simulink model "kuka_sim"  (R2018b)
settings: Solver=VariableStepAuto  StartTime=0.0  StopTime=20  RelTol=1e-3
model workspace (MAT data in the model file):
  F1 = sym
  F1.s = 'symobj::fromString("eJzVGktvG0V4/AiukzQE1CoUUtVQ4NILFMGhFZWD85CluAEaUIRUlo137Czdh7O7TuIgoYB4lQMcgN64IuWIVHHrtRI9cEA9wKXwA5C4capkdmbX8XietteNEksj7zc7833ffO+Z2QwAIA3A3q3wP5tJjYV/xadB9MuEz6fi53AMyKPmt3zd9826g7t73l9EbRuanlHY0j1TX7dgwdFt6BeaPjQKplPwW7a7/uF807ZbZQM6gVkzoQdImmkKZxa1DdcyqDEiHvF433IDqv8x1PzAsMx1TG8cdH8nUfNhcK1lz1mm7kM/WtsZgsY9YvzIBHYaNaFM+hPK83F/yEjxfPycooQ0jMAyqM27Ni0sLMiKHnjmDuZRRDNDPf9K4MhS8BhF43HUFnYaHgwF5zqLJkRLBcVnuvgw7XNdfIh+NnxfnOqi6cGJ1pQ2DdxP0p7g4KmEfRnA/Jh5JDwpMZgMxUsOtZLrBKG6Ed5n4/7psH0V8QAMic5OoKbBUEA+3OTpbaWJ8TJ6NvRA56yjQyfLw6WZNSAZE/Fi6bstzfUkPGO70eBmU7ewLGfjd6m4ZSiZp1BnO/xJ7GhG5SOO2/ApWjw8T6l8OFqf7mDzUenFgvEqGRokfFayrgJnLC2v7AC+Rq8/zfPpkt5oWC1mfTK/fZHDFx13SPng5jYYGozN2ToaVJzp4u7BSfJwgYJnOTyK4qBqbYzPhglkselUgYLmhIIOIxNOXJpWxJth4LPxM9JTJ+ZMEuvLR/x27KQbl9rtT04ANi7RMnuCWhu2iSDCxfRz8iHutwEjiwlJjCTHnVLI4NVHIFMV/EIXHDnufm1MVvyg5/E6dMKUEZu2XL9kvufiml+paNdW3y5fXcLvRTkxz7F3wt72RHmQ5oeEn+TZ007Ep0yWSfyXt+ZH7ccy+I0h5jM6rFSWu+WJWC8q3xtF3MU5tVQNq+R11xog5/WrP5xvdAPXSyRd3L9WWab7cR5YsKAd125MjWnj3UMi+yLhBQpeOmb2hDZIY296phPnAXLsODUW1e5TDtwOS9sAHoi41/7IPMT4usHSGJUdYnsIeQNAUXPqXt0HqjrY0506xLz21Lzp+B+I6501Cp7irJekJ5LpUbchEn5XYgP95siUQo603Eh9H3VZMfGS2IOI5NZvTi3x/AxvE+R+xvjFusvE74H2cr7roTOKGWIM7a+ymFtXyLFwzPSM42qoZz8+rOrHP3j+ItLHOQo2JTEtsrmmw9v3qvRC+x29ruOkExzbqy70qlFs76duKg3gR3nU0LHPxSCM5rhbKuskdUbjmMkex+sbEEWmnnFzQL5nwfUcqt/LV1fRO9F+JUfhle1XyHHzEp3QOjgt0Zer8KMpIK4ZRGcg9Djar7FsNAfW9QAZtHBei8PbMOfA3JqrVEUnBdyzIF4OIefjvBG0GpCn87AihXV80p6oVmfkRdgSbS+H6U/bCec3+swp3PpgFYOKfOEHdhCdX4vGRfZ3cHsitGmVXc3y7MqI7jY6OHLcPFTVfRitRRZnFyS83JS8+1riN6q9CpMXkN0tLq/MrbL80rGcpDNIDJpR+MrrktyFc6MHg6bnMPyheSe7YM+7b/uU7aDrkNaaNU+vctaaBr2/ywTPotj4vYQWtjHPbTqcfSst21sU/EOfNJPEX3wWVHWdLegFWuAqefxiwNgpm3vY9ccw8ZKJKY2NsExW3lPmLitw73Pe8+4o6fyvwimqbei98Z6Cn9U+c8M7Cp7eV7zXjoENkHCScwoS/kDxnneHe9TkQvoGrgnm8aPUZgMK3hqCruzuQjb3jALm0aK/fWD2gsSdCzn3yhDrIvw10TOJt0jBt3lrKJlG58yQuZ8HUezofIOSVsgE3d1NRzK5dKns1EzHDFoD5IgrgHPWReAhx/4yAh9g9hKGWasB8b6PqYNrGJTmRPYbjYiGSCYXODlbtu7rCXLyaxR855DjTlJ4j4In1bk59VBhB9gnTH8Xemw9NIo8fTdBnr4r0W2eo1umPifWJaotc8Q7mp88HSMy/HHIRsn9/HNdng++P8gQfbE/Cf0m2qvZTUv0rUE96j+o39vt9sfh32doHvrYrHr7m3tg76MyybuSXsNqxmeUIpnfB5x976b2smYY+Hs7kp+tDj/owub6w92XbvzzU+vnVz7/7cuNIKf4Duq+hNfovqnhbscfWjJ3HCE/gML3HsVbs8Mb+ljkvzv7/75V/rE+8d3+pzd/f/C3grc/FHyT8J8U/NcAcx8MIk8Q6ZeJvee1NY0X9xeX55b+B5OCZnE=", 2)'
  F2 = sym
  F2.s = 'symobj::fromString("eJzVG2tsFEV47q61FEoFA1QU5BQFExKNTfAHRNLSBzZpwUgRfOCxvd1eV+92r7t7bQ9fNTGK/JDEKJr4iD/0hzEmREH/+PiBIUETjYlIhKCJJD74gSGCBjHWndm93tw3szO3t0dDL5l0v9nZ7/2a2W0CIRRHaHK/+7chEWt0/3Rch7xfwr1e5F+7a1AzHnbRVmxbzxhkuuJ+Ox7jmm6pyTHF0pWhrJY0lJxmJwu2piZ1I2kXc+bQI92FXK7Yp2qGow/rmoVomnGAswGPETOrgjVBPJL1dtZ0wPxVeNiOmtWHCL25qPybj4etOVuLuc6srtia7cm2lKLxJbW+bgpbjEegTqpTys3+vMtIx0r/OgaUVIvCEnh0mzmoLKLIAcWx9AnCYxDNBLg+SuFoAHAjoHE1Hj0TeUtzFWcavbqGRUUd15fxEdoryvgw/Qb3fkdrGU0FTixTXFfJPE17HgfPgDuXQMyPeY6GWwQOkwC8NOHRZRqOa26M90Z/foE79ng8IFVgszl4pDRXQbY2yrPblgLBy9hZVRyFI0eJTgMPV0ofRoI1Hi9ZZXcxZVoCnonfpLTRgpIlulzm34v5IwF0HsOTU+5P4EdtshgxzLwNaPHwXCuLYU8+xSDuI7NLVvOlZGjQ8HKBXEnOWqivhhCxBuWP82K6S8nns0VGPlHcruLwBfMOrR8yzDxDg/G5nIIXdbSVcVfgpHlYA+BlHB6D8qBMNiZm3QLSWzDSSEJznoQOoxNOXlogyTe1wMv9a2ynUs5poeRr9vgt+Uk5L01NPT0HsXkJ6mwhkI34hOPhYuY59ZDM5xCji3mCHEmvWyTRwdrLoFMZfEsZrDvuan1M1Pzg67kZzXBLhu/aYvvS9Z6Lq3vLQGrr4L19mzeR+0E1sZnj75S/TQbVQcgPDV/D86cJj0+RLqPEL0/myx3HInhjDc8zNhwY6C+3J8F2kcVePfIuqaldabdLHjKzIWpetfYj9UZRSb9E0yXzOwb64TypAz1ZLef3bkyPmSO7h0j+RcM9AN40y/wJb5Aa77F0w68D9Nq5YC3u3VsNbdxtbR1tWsWV/kfXISbWVZZGvfyQ+IPLG0KSnlOxMjaS9cGWYmQ0wmtFzxv3/6LgfmcHgFs58tL0gnR6pfsQDd8n8IFqa2RMokeoN9reV7qumHxJ7UGC9FZtTe3ixRnZJojjjImLIZPJ36H2crZp4TOKNmoNjFdRzs1I9JicZXYmedW1s+0fVlUTH7x4CbLHCgDrgpzm+VzB4O17ZXaBcQflmk02Ibk9bWpW2svt1fRNXSHiqBkPfOzT7rjZnEwLdR2lz8jPMt2TfP2ohjNTxbpOJN6zkH4O9+99mwfxvaD9ShPAK9qv0Ou6BTaBNlgssJcpiaNWFNwzBJ2BwHUwroluUoaWURzs0IHPFTm81XIOzO25utL4pIB7FsSrIfTzpG44xbzGs7nbkWoZctIeqVdn9EX5EvSXmYyn8YjP56usKdz+YJCAknphOznHO78OWuf53/Tbk0CflvnVMp5fqd67jRKOJm4dSiu25skiyrM9Al6eF9zbK4gb2V6FqQvY73r7t3QOsvzCXE7TCZOD2iSxcpegdpHaaGlOwTIY/vBz88tgxb19Veo2rBzCXnPYUtIcWeOo8ree4jkoN74koEV8zDILBmffCnW7H8AvV0kzSv4lZ0Fp0xjTLCflmFIenw2ZO0XPznT/UUu+ZHJKfsRtk6XvKZvWS3C/y7nPe0cJ678MZ1BvA/fGkxJ+BqusDdskPD0suZ+aBT5Aw1HOKWh4l+Q+7x3ulaYXOjZIT9BNLoU+6wB4rAa6oncXomeXSmAeLfjtA7MXpN650M9uqEEuKl4jXdN4OwB8kCdDl66WzgyZ9/PIyx2lb1DiEp3gd3cLPJ2sW9dnDOuG7hRD1IgNiHPWReGh135Uhxhg9hKqPjyMgvd9TB88TEBhTWS/0fBoBOlkDadmi+TeGaEm3wngT2c470SFJwHcIq/NsX8lfkBiQrd3axbbD9WjTh+JUKePCGzbzLEt059TcgX1lk3UPchPM8wRCf467KP0fv6mMs/T3x8kqDk/niR7tXy24J8ZBn2r5K3LFbKcbxLIXnM01Z5STQcJ9Pid4N4xxHmHMJq6A+Jj3wflzXHJh5AEl60bkG+fBv72soKXBwS18BiAT8jopk0b4sfPTO+HpqamnnD/POOOxjmI/fnfcdHrHy+txx+gnDq8Ob5w4oL60M49B8+Ovb4KfPcl4//7CPaCMtHwyRA8HAfwTxxctPwTiNLXt489ePyzg/s+ePOV1emRtQdeqUJ+5jzF9bOUSpyX4aNquqgyzmQyn5HIKLQxoNVYg37rZXOa590lnnHSf3tPy3sf//7Nk7teuOHzX7bbkyH1w+OZpuWUaOGXtPqPo3uPHt74/uJLX5398Ix9yKdFr3+qtN5NtOiANRJ757Uvkl//vfX0mueW/ICi6fPkZdJnocQz/qj37ot9h25dfWLbG69eGDp3W9s5FE2f0N+E+uTkIKE+QQzC8/8wdcCPz3ZefP4WMs/R8M9AnnFExfb2t1bfnlz6ycVTS8aG7j+75MWQORXmwj8BfClEfiK9cIaAwhx5vo65R6gLNDOxErVm/BUxNmj4D4H9wvo2Df8H4NMR/PnXShj/c0XN/gB0iV2wZt//p3Y/jUH9QbvQuGqpgTQt2OOfR5z95crUDnyuxuxte/s7N/0PY1GX6S==", 2)'
  F3 = sym
  F3.s = 'symobj::fromString("eJzVG21sFEV0rtdaCqVWEQEBqaL+URIpIAlfKbQFG6igFEJM9Nzebcvi3e51d49yqAQTQoREiaIEfxj9YWIg4YfGkBg1MTEhwY8/xg9UQDEYlagQSIwose7M7vXm3szO7NwehG4yuX2zs2/e93szs5dECNUhtPOA91ufTDR4Px23If9Keve3BPfeGNSEm1N0NMcxBk3SXfG8Hbdh3bAzbVs129D6s3qbqeV0p63g6Jk2w2xzijmrf0tXIZcr9mR00zUGDN1G9Jx1AGc9bputbAaMCaORjHeylgv6b8DNcTNZo5/MNx6Vr4m4Obq7vphbnjU0R3d83qZRc3xCja+ZwCbjFiqTaEK5K+j3COmYHdwngJCqEVgSty4rB4VFBNmrubaxjdAYNmcS3B+ncNQDuAHMcSNu3dvytu4JzjJXGjpmFXVML+Mjc88q48Pz13vPO1rKaCpwYp7qjAzpp+eewMHT6/UlEXMx79Fws8BgkoCWRtw6LdP11I3x3hH0t3rtOZ8GlBHobBxuKd0TkKMP8fS2tkDwMnrOaK7G4aM0Tz0PV8oYQIIxPi1ZbXsxZdkCmondpPShgpYlspwRPEsELQlknsCdI94lsKMpMh8xrbwD5uLhmSrzYZ8/zSTmI9NLVg+4ZOag4ZkCvto4Y6G86hV8DfJfx/PpTi2fzxYZ/kR+ew+HLhh3aPmQZuWZORiby2l4UMeUMu4KnDQN9wJ4BofGsDgo443xWS+BrCyYaSSZc4JkHkYmnLjUKok31cAzg3usp1LMaab4a/LpLdlJOS6NjDw7DrFxCcrsJsAbsQnXx8X0c/Ih6c8hRhYTBDGSHneLRAYLroJMZfDdZbDmuKPamKj4wffjB3XTSxmBaYv1S+d7Lq6utb2p9X2P9Dy0ijwPy4lNHHun7G1nWB6E9NDwzTx72ubTKZJlHP/l8Xy1/VgEr6jifUaHvb1ryuVJuF5kvleLuEtyamfaq5L7raxCzouqP5JvtAypl+h5Sf+m3jWwn+SB7qyeC2o3psbMkdVDLPui4W4Arxpj9oQXSA3rbMMM8gA9djwYi2v3FlMf9kpbVx8VcaX90XmI8fUMO0et7JDYg0cbQpKaU7MHHSSrg23NHNQJrRU1b13wi8LrnU0AbuHwS88XJtPr3YZoeKPABqLmyIREjlButL6vd1kx8ZJag4TJLWpO7eT5GVkmiP2M8Yt+i4nfSms5x7LxHsUUagz0V1HMHZTIsW2M6ZnEVU/PTrBZFcU/eP4Spo9ZADYEMc23uYLJW/fK9AL9DvI1lnRCYnva0u20H9uj1E2dCn7UhBve9ml3vWhOuoWyjlNn5MeY7Em8flLHkali3HIkXrOQeg7X7z0P9eFnYeuVRoBXtF6hx3UJdAJ1MFmgL0viRy0ovGYI2wOB46BfE9mkTH1Qc7FBh75X5NBWzT4wt+bqTOOdAu5eEC+H0O+TvOEW8zpP515Fqg+SnfZYtTojL8qWoL1cS38ajvl+PmJO4dYHfQSU5AvHzbn+/nXYON/+Rk9PQm1aZlczeHaV8c82SjgauXkorTm6z4soznYLaNkjeLZX4DeytQqTF7DdrVyzdnkfSy+M5fQ8KjFoisRXlgpyF8mNtu4WbJOhD783sQxWPNsXUbaqfAhrzQFbS3N4rUOV12KK5rDY+LJgLmJjtlUwOetWKNsDAH4l4pxx4i/ZC0pb5lbddlOuJaVxt2LsFL17reuPauIlE1Pym70yWXpO2bhYgvsQ5znvjBLmfxnOsNoGro13Sujpi5gbNkhoelzyPDUGbICG4+xT0PATkue8M9zrTS60b5CaoIvcCm3WBfDWKuYVnV2I3p0mgXlzwW8fmLUgdeZCv7usCr4of411T+PtAPC7PB46jUxpz5A5n0d+7Ch9g1InkQk+u2v1ZbJoUY85YJiGW1TIEcsQZ6+LwkOPPVoDH2DWEhljYACFr/uYOniAgMKcyH6j4c8RJpN7OTlbxPdjMXLyAwD+8BrHnbjwTgA3y3Nz4orEDohPGM523WbroVrk6WMx8vQxgW6bOLpl6nOKr7DaspF6BulpgjEiyR+HbZRez99Zpnn0+4Mk1Rf40+i8zYi3VstnC8GeYdi3Sv64XCHrVo6DdTmhwzHImpPpH0rNQwI5fynIQV8hzvp2KNWeylhuVJzwGcQZ0DgX4mPPoPLWMOfjSxr313zc+DvPinGPSnim4ZMyuactB+LH74yuvUZGRp7xfnZ5rWEcYq/gm7HI41Glbcl0RnKOJ99UhiitYuwpAP8E6CiU6PCcHr39Uve61eOaH3xx0sn/Pp+45EgEOsJs4HsAf8fRDw2fBnQ9XaILf3j5xq5Xj95/tPXs6wsnH7pv0o5D4Bs8FbpkdiuyC/rZjwD+RsHeoCygjk5QuBpi0P8NkCn+7GTU5i5ruy6Yu6dfeL94uHPCwY+i6FrEwxkAX1L0Pxo+D+geLtGNN2S0PY0vH31v7tIvFuy33lh7tgfQDeVVjexp+C9Ay44SLV5iQWcvzvri9NDeFz5eccT499M/jyM1vw1i7TyVWCuT5YmIeKLYflSblMn4fISYRMM/K/B7XsJvmI/K+JfZN4yj+JCH2AUuzN6e33/51h+WTT75fHLXr38fPBwhXjF1+iABhTT8o54j2nk5AvqbMCdE4IWCE7DGO6EiN6QWk2i6ahk3XUT5/FvHVi+c885r56fWb2zZ8oG7X5FGiV0lWhRw8XwUxq5a+mzkmBzYSJit8uQftY6APMM64g/F2EHDvwFdNCvgulKjuAtpEv3XgBf7afphzXKOwgXXeCr1fBBL5nFiSWL8VfDXauqHWvpU5BoKxMZa58lLMXBL6hwio8h1jmIOgHZ4WTGP0fC3NfIzqOdTtYvhjKzPKeAGez2J+rB8ie3vjqUHNjzauuThxu4zM3v2vYmfqeSiXyS5SMGXo+d5Ht1q9lRR88GxKnHjWwCfBTQ/VaIZ/yHlM+r63GuKNENZw3wqnAvFW+NAW4d6ng/gexT4OhFRFxJ/hPaTaFd4F34HdUpBVr+r+XIsWcnqjftj5Gcaz+0AVqljLoJ3744Rq2E9KuJXMYck4H87VHMIjQucX+A/UNcshirInomhsI6ZU72tJZbUTo+JhTF8AOa36RybYM6fZqc24XN35uxr5Zrlq/4HI4LjiQ==", 2)'
  F4 = sym
  F4.s = 'symobj::fromString("eJzVG2tsHMV51ufgOC9CRWLSBOE0KRTSFyYgNTxkc06iUJug4KIQ2l7Xd2uzcLd72d1LfOGhRFQVkCr90Tbwt6qEqPqrUB4C8gspVau0AolA0qqNq0SN0lZVVKmoSCCzM7vn++6b2Zmd3UsUn7Tyfrsz3/s1s+MCIaSHkINHw7+9BWNR+Gf4iyT6FcL7a+P7cAzpp5ff9E3ft6cd9rjj/RC99lu2VxncZ3q2OVm1Bh2zZvmDDd+qDNrOoN+suZOPjTZqteaOiuUE9pRteQTS7EE4e+n1qFutoDFJPLLxftUN0POr6OUHlao9yegtIe3fcnr5VvBgszZStU3f8iPZ1gAafwDju6awVfRK1Ek6pWyMn4eMDG+I7w2kpCwKK9Br1K1hZTFFjpuBZ88wHpNoFtD97wGOXgQvQjSuptfWmbpnhYpznW22RUUlw2vb+BjtG9r4KP3e8P3wijaaDpxUph67wp5D2ksFeMbDZwXC/bh5EF4mcZgC4qWPXkXXCUJzU7zr4+crw+vZiAdSkdhsMb1KVqgg39orstvOBsPL2bliBqZAjhadXhGukj1FJGMiXqrmgWbJ9SQ8M78pWXsbZpXpcl38zoivAtK5QR/OhT+JHw2oYsRx6z6iJcJznSqGI/lMh7mPyi5VK5aSowHh6yVyDQrGYn31asQalr9HFNNFs16vNjn5ZHF7o4AvnHegftjl1jkanM/VTDpoeKCNuwMn5GETgtcJeEzKgyrZuJgNC8i2hlMmCppLFXQ4nQjy0kpFvskCXx/fUzu1cs4yIF9/xG/LT9p5aW7u0GLC5yWss2uQbMwngggX91xQD9nzGuF0sVSSI+G4axU6uP0S6FQFf7kNdh13Wh+TNT/0fsm05YQlI3ZtuX1hvRfiGt05XnpwYteO+7ez90k1sV/g78DfDibVQcwPhL8g8qeZiE+ZLvPEr0jmSx3HMvjeDPM5G46Pj7Xbk2S7qGKvG3mX1dRiOeySJ92qRs1Laz9Wb8wK65cgXfZ89/gYfs7qwNaqVYt7N67HrLHVQy7/gvBWBG9fYP5EF0iLHvBsJ64DcOwSNJb27isca3/Y2gbWvIo7/Q/WIS7WKzyNbvkh84eQN0IUPafpTftE1Qd7pjNtMV47et6e+C9J7nd2I3iFQF5IL0mnV7oPQfghiQ+krZGGQo9Yb9DeV7quuHwJ1iBJektbU4uiOGPLBHmccXEx6XL5W2st57se3aMYAGNwvMpy7rRCj4MLzM4sr4Z29uPNqjTxIYqXJHvcgGBbktMin2s4onWvyi447rBcC8kmLLeXXcsrR7k9Td9U1IijfnrRbZ+hIMzm7LFU13n6jPoC0z3L149bNDN1jBsh8jUL6+do/77j/gn6Lmm90ofwytYrcNyoxCbYBqsk9nIVcbSCJPcMSXsgeByOa6abkmNNmwF16MR5TQFvWfaBhT1XsUx3CoR7QaIaAuezuhE065bI5mFHak2znfZcvTqnL+BL2F8uZzztzzm/nrKmCPuDCQYq6oUf1IJo/zppXOR/819PEn1a5VfrRH5Vib5ttHD0CetQ2fStSBZZnt0q4eU5ybvnJXGjWqtwdYH63baxnSMTPL84l0M6OjloQBErd0tqF6uNnhU0PIfjj85b3gY73v0kpW515ZD2mlOeWRbI2kM6f3cCnpNy488ktJiPeW7DEaxbsW6PIvjnKWnmyb9sL6jsOvssLygFrpLHH2nmTtncy91/ZMmXXE6pPxq2ycrvlH13KnD/SvBe9I0S138VzqTeBq+NDyr4mUhZG76j4On7ivelBeADEM6zTwHhHyjei77hXml6gbHBeoJRdiv12QDB+zLQlX27kM1do4BFtPDZB24tCL65wLn3ZJALxGuue4h3GMG/FclQtCutPUPu+zyJckfrDEqPQif0293KSCdbtuxwpmzHDpoaNeIeItjrAnjg2Ne7EAPcWqJiT02R5HUf1wdPMVBaE/kzGhGNJJ1sEtRsmdzfy1GT70Dwscucd/LCBxG8TF2bjU8VfsBiwvYPWB7fD3WjTh/PUaePS2zbL7At158DuZJ6yz7wDvPTj3NEQTyO+ihcz3+pzfP8+YMCeBbH0zxd8Z5hvdqI9wyTzipF42qNatA5DuvqA0kdOUmS+3nGv2+ztSr3fG9pc1qa+N1JMb4hIrHTh+I5t8E5i9LRuRXT4caUXar5Dlx/VvAG4dMErK3m5uaeCv/8kPK3mPC/+ExY6vGk03dU9oTv/obgjxT2S5JfZE8I/1WDh9MI/juYe5WmT2HZoE7psQmmU7owv+mY++T6Xz9y96t9ew4dKr68C53LE+kUwqcQfDaJVphAyHfX3nL8lRdPPfnBGycuVC4UBzRpYf2c0ZGLqH0Fwv9A8AUduRAtUSxiH4HwLIL/guCLiJenW7zQYva7m7d4S197qfmNt2+6+r2TD/07g9xJY1W5k9vfC3NSqeKysxRZ87FMD2cRfE4D1xmBfXHsJcWiKoez3jXM4aUKE56TQYfHrHoT2GJIxxY6eU18DqLu7o//AUDm23tyxP95hc1U/iCw2a0im2GeRXRgPB4goGa9PLP8Tw+885Wx684ffuGZWx4eIXrxiPKrsQTR8iCtnw68deTcJ8+6J766ZuiXv/jNO5r5VRX7An3d1tJXWhqyM986/od9YVaDB5xvsR/NasY+tA+u0+d17EXy+cYqBMv2TBJyxOZu5ohTXcKDa/FZTR5wntehm6YWpum/MvqTsOfJ6uezglqUOm/p5RIDfofqZu9aJ6DHO9LYu/bYrqPrN19zx10/vu+f8bo8c4+H+4n/5qhNuDeV8p2z58a9C+S7y72ncTPR6D015ZL5tk6fOId47kU8P9Himf6DxAnw+2N4afo59u1ZHVok3zpB0Q8ZQwj+uoZcay5N7jZk36dV9W29II/C98s1cMv6cB35PkM8fFMxl9tHnmZgYi8j8okE/AbGg/1lj9xfcOxL/WeZps4EveNmQa9trNa0IZy7ODsuzrf+h+CPM9Y+bD+dPKaqTxdz1AyEi+X1PHsjENeNOfjCtexidjtwuQevneiBwvnc/PFzxXdXn924+r3Db/xn5s33D5Pu9uLjmri6kXvRHocxnCO28P/X4dyrW1sgvEHHLpo9xWcKnejUjDx7Y5Am+kZsoG8oLO+mxXWXIqer1hppawnuNfYIeM4ap/+/NP6utU7Ee4s4p8Faolv7IB50Jly5Rtepdxq4cL0zvpbDfqI9qqy5D+dsnEcncuDalUNGVR7ZqIHrX2jut7PzxeXSb+WsO3DuIzljGuJC570M/J2XnY/YUNpNx3FnM7aNjWz/HMzJdIk=", 2)'
  F5 = sym
  F5.s = 'symobj::fromString("eJzVG1tsHFf1jteJH3kTB6ckpds2gEQAKU5cqQ9HDnZspbIbSN0qCirLeHd2O7A7s96ZTbIpD/NQaSACVaIRH3zQByAkFPHRVlWlSP2hKhUVP7Qp9KW0qAiKiFokhBDCzL0zm7177pl75+5Moni1Y8+ZuXPOued97tzNEUL6CFk+G/zvzxlrgn+THyHhJxecj0TnwRgyRA+v5ZmeZ1ccdrnr/hg9Tlh2o5Q/bjZsc7Fq5R2zZnn5pmeV8raT91o1d/HL081arXWoZDm+XbatBuFp9gGc/fS4362WwJg4Htl4r+r64Ppaenh+qWovMnrDpPPZQA/P8u9u1Q5UbdOzvHBu13E0XuTGZyawbfSIlUkyoeyKrgeMTN4cnRtASL0ILEePabcGhcUEOW/6Dfsk4zGOZg6c/5bD0Q/gNYDGJnocPFlvWIHgXGfGtuhUyeSODj5G+4YOPkq/P7g/ubGDpgsnnVOfXWLXedrrEDzzwbUcET7Cczy8XmIwOcDLAD2mXMcP1E3x3hhd3xwcD4U8kJJEZ4P0KFiBgDxrCdPb4SbDK+i5ZPomMo82nX4MV8EuE8mYkJeqeapVcBsSnpndFKylplllstwZ3TOiIwdkbtCLK8FHYkejKh9x3LoHaGF4tqt8OJyf6TDzUemlakWzFGjw8PWSeeWRsVBe/Rq+Buffh/n0lFmvV1vC/GR++3GELxh3ePmww60LNASbq5l00ORoB3cXTp6H3QDeifAYFwdVcxN8NkggM02nSBQ01ynoCDJB4tJmRbzpBb4+Oqd6asec9dz8hkJ+23bSiUsrK98cJGJcgjLbAubGbMIPcQnXkXzIrteIIIt1khjJjxtRyGD8CshUBX+sA2aOO6mNyYofej5csZwgZUSmLdcvn+9RXNOH5wt3Lxw5dNcsux+XE4cQe+fsbTkuD0J+ePhDmD2dDPmUyTKN/2JzvtJ+LIM/28Pzgg7n5+c65Um8XlS+l0XcZTl1qhhUyYtuVSPnJdUfyzdmidVLPF12/ej8HLzO8sDBqlWLajehxqyx7iGVffHwQQDPrjJ7og3Sms81bCfKA/zYYTCW1u4bHetEUNr61mURd9sfn4cEXy+JNLKyQ2YPAW+EKGpOs1HxiKoObphOxWK8dtW8fdF/El/vHAXwRmS+PL04mV7rNsTD90psIGmONBRyhHLj9X2ty0qIl1wPEie3pDl1CvMz1ibI/Uzwi0VXiN9avZznNugaxSg3BvqrLOZWFHLMrzI9s7ga6NmLFquS+AfmL3H6uAHAtiSmhTbXdLC+V6UX6HdwXqtJJyy2F12rUQxje5K6aUrDj4boQZd9xvwgmrPLUlmnqTPqq0z2LF5/xaKRqWvcASLvWVg9R+v3Q3ct0Htx/coAwCvrV/hx0xKdQB1sk+jLVfjRRhJfM8StgcBx0K+ZbAqOVTF9atCxz7UQ3npZB0ZrrqkiXSlA14KwHMI/z/KG36pbmM6DitSqsJX2VLW6IC/OlqC9XE1/OpHy+XrCnILWBwsMVOQLz6/54fp13LjQ/i6/PYm1aZVd7cTsqhS+22jjGEDzUNH0rHAusjh7UMLLacm970n8RtWrCHmB2t3M3OEDCyK/MJbzdHRi0KjCVyYkuYvlxoblNxuOwB99bkMH7Lr3w4Sy1Z2HtNYsN8wiMtc+0v25neM5Ljb+SEKL2VjDbTpI3wplexbAjySkmSb+srWgousctxp+wXeVPD6oGTtlz17t+qOXeCnElPr9QZmsfE85cLsC9y+R+9g7Spj/VTjjahvYGy8r+FlImBvuUfD0RcX9wiqwAR5Os07Bw19S3Mfe4V5rcuF9g9UE0+xUarM+gI/3QFf27kL27HUKGKMF9z4IvSD3zoV/dn8P8+L8NdU5j3cSwE9ic5iyS+01Q+H9PAljR3sPSp9CJvTd3eZQJrfddsgp247ttzRyxH6CrHVxePixT2fgA0IvUbLLZRLf9wl1cJmB0pwo7tEIacTJZDeSs2Xzvi9FTr4FwOevctxJCy8DeL06Nxv/VdgB8wnbO2U1xHooizz9fIo8/bxEt0OIboX6nJtXXG05wN2D/AzBGJHDx1Eb5fv5mzo8X95/kOOuRf50me4GgvVq9WozWjOM26sUjqs1q373OFiXMz6KLsUmXl8qjEMa/Nz+INHByxK5voLT2peUFrz3MkF66aXC3kLJ9YmERxVOqcw8m/XpyDz2JqWJyQzBR/eado17k8OxJhmOPUShDx5+QzL2dQC/RbhecWVl5WvBv+9QvgaJ+In2uCUeT7p9AdMRD7+tkHvcHDE98PBFDdm9BeA/I3BS/bOcH+i/UGKGHGsDaeWi6VdjOn6lI1v8/XHdPRFtnOafewfAxzTkAXX0V4XO/qIho0hnezCdQZ5ldHTiKfTJPyriKMLv3ja/SWX4fkb6h7p4R4OHiwo9YvJOyte/EdyafrIvSz/5X0Z4/gTgdzV54OH3NOn2WkdA2+5Vp9DW3lboVGZr0LbeRPji81zQ33fy3AtPPjzzmZcGX3xm4ic7tg/vfYGo81xS37/QDRtbAR/1Nh9BMU5O//3bn7p05ulPTj+0u/LYhufWgj3oKpm8yo2FdUhMnNmnG2egXP+jGZt5+BKi/15t6bWM/BHyoOOPUDbvAd2PJpeN8WEA53XsN4HdIPFxPMv4+KqEPqz9LmjYDIx576awGRh7NeIn009WcuLxDmvywMObAHxTwhiWgn+Bh2ENXcK5b5Locm0KGV8AvkONnPnOUPDnjYH8U7P3bJ0+/8SeY/aR4WeJXo+D2WNiWnrxHZU1T+tUmxZ9oblt/McPPvqNb32fbP/9T2d/9ZtfaOYSzDd42mMp9ZyYbxLqgx//dX78xPCFx4NvPfhOPFGfGNacZ1Z1nKx20cFzCcz1gfZc6Y9lfsd9XgoOxW/UYJxn68IVBsbW+Nj6RRz+DwAMa7JjAMb6gcRzJXp+KevHVT02D78P4H8BW96vgQv2MKBmNaYUepDJWtFDG3CvH6yHpT5FtGRv7L5CcdvhefxBc2nH+SNnb9y35ZY7ztz5t/4e/F4Wt6W09OSB5ngevjXDuHw4RT6B9cOtAJ7XwC2rY3T8D+uPY2PGudmLp4LvSPA998DIOfqLqDS5HMoW7Ns37lDgzqq/TjxfTR/A+m84317jkaIfF2QJbU8lW37srmxsTfCHT4DxOr0t9Hn47hTGX+k6ANGz46RrOyp5wH3R/5TkKxWuSXl+UvZtSWsQaNPHEJ7j7Gy9pp8i6ynjyDqzUdbQHbQbuF70VcLZSe7x17+77R8//9muM7/+YMsrm8sp+4m8Di2iVxPsAvCnAexp8t0eO9h7bDXAPpuueNdrv5x2/UInxihqAfg+w/hCClqKdb8u2WmuuxhzGnwo1gyN+zT4ALowqhp8vAae/agiv2nkM8FGwL4QrXVEkMMMsP9Tp6YT9AZqAp0419UjYGvVWdXWGusU6PoKD2vU1qq1LePzKfiCuMZS6JRfp4W/M0pTp0ObVcVWmV9CO9PAZYA5GWAvpk68MMA+P8PUmBOMU3cisbrHWGzA38/BuK/Ttw1I5JHivabWujDUP7YuHBcPdWs4Hg/4nZsxksJHtwJ4SWP+MHbkM8S1nCJWqPKS6n2DTi7RkT3McfemsH+ox4dT4II1rwVgnZoXxrFHepe9sQfAp5E5CnuDby4cpb+JEPYlz8wdmP0/qpZvwQ==", 2)'
  F6 = sym
  F6.s = 'symobj::fromString("eJzVHG1sHEd11ufEdpK6IXJkQhLFbdoI1EJVJ46gUSK7tmPSxk3UmDQEwbG+W1+X3O2eb/ecXCKiVEIRRQIEpVWKkCg/+EGlVqpa+o8fCKlSKfxBlFYtpAopKoqiUlokKGkxO3N7vrk3b2d2dtdRfPLq7u3Ovnnzvt+bXecIIV2EnHsi+O7OGauCr9FPkeYnF/weCH8HY0gfPbyGZ3qeXXLY6Y7rw/Q4adm14tCCWbPN2bI15JgVyxuqe1ZxyHaGvEbFnf3GRL1SaRwoWo5vz9lWjfBzdgGc3fR42C0XwZgoGtl4r+z64Pxqenh+sWzPsvnWkPbnJnp4ln+kURkr26Znec21beLm+C03PjOGbaRHJE/iMeW28HxAyOj28LcBmJSEYTl6TLgVyCzGyGnTr9mnGI1Rc+bA75c5HN0AXgXmuJkek6eqNStgnOvsty26VDK6uY2Pzb2tjY/O3x1cH+1vo+nASdfUZRfZeX7utQie6eBcjggf4T4eXidRmBygpYce467jB+KmeG8Jz68Pjm83aSBFicx66ZG3AgZ51jwmt0N1hleQc9H0TWQdrXm6MVx5e45IxjRpKZunG3m3JqGZ6U3emq+bZcbLLeE1IzxygOcGPbkYfCR6NKiyEcetemAuDM8nVTbcXJ/pMPVRyaVshasU5uDhrZJ1DSFjIb+6NWwNrr8Ls+lxs1otN4T1yex2B0IX9Ds8f9jhVoU5BJ2rmHTQ6GAbdwdOnoY7ALwFoTHKD6rWJthsEED2150CUcy5VjGPwBPEL61X+Jsk8NbwN5VTy+es49bX16S3pSdtv7S4+EgvEf0S5NknwNqYTvhNXMJ5JB6y8xUi8GKtxEfy4wYUPBhZBp6q4NvbYOa44+qYLPmhv9eULCcIGaFqy+XLx3sU18Sh6fyRmQcPPDDFrkfFxD5E3zl9OxcVByE9PLwB06dTTTplvExjv9ial9uOZfC9Ce4XZDg9fbCdnkTLRWV7WfhdFlPHC0GWPOuWNWJeXPmxeGMWWb7Ez8vOH5s+CM+zODBZtiph7ibkmBVWPaTSLx6eBPDUCtMnWiCtOlyznTAO8GPXgLE0d+93rJNBautbSyzu1D8+Dgm2XhTnyEoPmT4EtBGiyDnNWskjqjy4Zjoli9HakfN2hd8kOt85BuB+ZL38fFE8vdF1iIePSnQgbow0FHyEfOPlfaPzSvCXXA0Sxbe4MXUcszNWJsjtTLCLWVfw31q1nOfWaI9ikBsD7VXmc0sKPg6tMDkzvxrI2QubVXHsA7OXKHlsA7At8WlNnas7WN2rkgu0O7iulSQT5tsLrlUrNH17nLxpXMOO+uhB2z7DfuDN2Wkpr9PkGdUVxnvmr09Y1DN1jBsj8pqF5XM0fz/wwAy9FlWv9AC8snqFHzchkQmUwUaJvFyFHfWT6JwhqgcCx0G7ZrzJO1bJ9KlCR97XQGhL0gdGc67xAu0UoL0gLIbw97O44TeqFibzICO1SqzTnipXF/jF6RLUl+tpTydT3l+NGVPQ/GCGgYp44fkVv9m/jhrX1L+l3ZNInVbp1RZMr4rNvY0Wjh40DhVMz2quReZnJyW0PCq59h2J3ahqFSEuUL3bf/DQ2IxIL/Tl/Dw6PmhQYSt7JbGLxcaa5ddrjkAfve+mNthx7fsxeau7DmmuOVczC8hau0jnZw9Hc5Rv/JFkLqZjNbfuIHUr5O0TAH485pxp/C/rBRVcZ8Gq+XnfVdJ4XtN3yu693vlHEn8p+JTqw0GarNyn7NmjwP0L5Dq2RwnjvwpnVG4Da+NzCnpmYsaGLylo+prien4F6AAPp+lT8PDXFdexPdwbjS+8bbCcYIL9lOqsD+CFBPPK9i5k925SwNhc8NkHoRbk9lz4e/clWBdnr6l+83hHAfwCtoZxu9jqGQr786TpO1rPoHQpeEL37tY3eXLPPQecOdux/YZGjNhHkF4Xh4cf+2IGNiDUEkV7bo5E131CHjzHQGlMFJ/RaM4RxZM7kJgtW/dXU8Tk3QD+1XX2O2nhcwBep47NxkcKPWA2YXunrZqYD2URp19KEadfksi2D5GtkJ9z64rKLXu4a5CePugjcvg4qqN8PX9rm+al5w9y3LnQnpbmxXuG1XI97BlGPavUHFepl/3OcTAvZ3R4Nqs5hfPz+d38vavA2v5IkFp3Pj+SLxbZM3ZR8elVCc//hNOxC64V0iGbS6iz5/M784zEaB1S4dSkf2fcueA1SH+Ijz5/2jHuokROETjuJkShFwXXg/P8RbF2Hn6LcHXk4uLiN4Ovb1H6eon4CZ9/iz2edNoJJiMevqzgf9QaMXnw8CUJP/6K8IOH/4bAcfUgtLXhlq1F6UJavmja1bCOXenwFt9brronw4eq+fveBvBxDX5AGV1RyOzvGjwKZXY3JjNIMzaPjq7E1ck3FH4VoX9nHP/Ow+9npA9QNm9r0HBJIVeM/3Hp+hDBrWk3u7K0G9lzxLp4ePgdjXvfBPBVDVm9qdDJuDS8kUKmUNcua9APdQ3q1sUYcYCPg3SjbykOTp0/8evth3+64d383oGn3TrtJaviYFJdiOtDXtPwIWHuMUI09QHqYVK5Qp2+qnHv68vPSwM8O2/IalhVHirDu567d3UKG3sN6Cp9iIjpKi0k7WsPHR3rv+/CD9YU1l74b+MI0crZDLAHY2yOmos++DV16fRA8Pds8DcV/F3SnGsbwvfY6wLvbqjm2orIgodv07CN18G9twB4B1jH2dY6qON4+Tf3fnfjtVfeff6K98u+D58qxeAZErt2Zxi7jMGYeHT5shlcV+VtMj0EPO7wP3HokvnKuH41jv4m9JEq/WS843WKFolLOvW5j049uefiW//7zFP/md75kwu0v6Njh3ctk/yHM5Q/7BVuIhrxWtNXbOPG9mraFZK772rl7jy9Z1r00hdkAtd5uuVLzwSOlGSTX6SN8RryQmN8XFvQoRnLj3nZjaVY/1UEV1J+wHzzmoTO61VbyPJpHTzvyXT5d9zn98GheMcS2gzb1ygxUMjnZb22KPwfABjWCccBjNWosddK9Ppjsp6Rjk28D+B/A127XwMXrKtBHWUcVshBxmtFn4fhThrj30N0Pba/jaGj0G9kIDfjELj+LwmvVbjgPhDWQ4tT06jsB8rweHKayZ8z9GswJsS9F/ppRQwwPqshk0HJWB092RoTj24d/rGmzvM0rdagvzcjOUMaVHW6ZO1Cfq27LxCVL2L7dfzYUc34IMkhtPIRzD8mXC+zW35NluJepH4dybJ+hbXTZk3Z8TCs5Tdq8BjWP2cA/AUNmxnmxmbZK6I7N0t1UunsSM8zG+7sf/TKM4+MvzOyQPTyF0W9b+zQWK+qFySlO+Ne0FlNHw/1J3a/LKQ7aXzh4wJ8fyRNTfUxEgMT1lTG6uS4DFB703/d0AF/RcPOJyXzptjf6KBBd5/zsoQ3urm1Yr9DS4aQrocksUIzhhkPIrhi90o17Rza5gDR6KGBudZp6gzSB9qN7EHrxATB38L1LPXAAudJntvwwdUX/3Di+X/sevKfvUdffYWk682D98OMxzXlIMuPkvqWLyfXS9irNb4Ixuv0Kr8njydp+mgGfBYbPJNgPJYi7kFd1JEp6Mcad6ag6y4A79XR65Q+AeZoP9bAtSDxATr1HbS1NPsmUMbYvkka/7Mc+XopBa9+mKF98Dl3Cj+F7qEmzC+VOfanU9AFa50s90DPApjPa3VjKY/nAoD3ZRjT0tR6P1tGv6xBl+BLP5/cvynrWR1fuR3AL6TgF3hvx3g6hU5Am3hWordJ8k0e/nmK+Hoe4Zfwbsf2/DH6TpvwXsn+g2NT/wcyZPj9", 2)'
  F7 = sym
  F7.s = 'symobj::fromString("eJzVG11sHEd51mfXdv6ctGlDqNuYpPDSCFEncdpGLQ62YxnZiSFuCJXgWN+tnaV3u5fbPTtnq22oqlBaiUoEDO1DeUBUgoeIhxR4gCekolIQVDSFAqFKQ0tLVFD4EaUCmZ3ZPd/cN7MzOzvrKDl55ft2Z7//v/m5HEKoDaGTS8H/9pzREfwbfD8KP7ng++boezAGdePLq3um59mzDrnd8rwfX/OWXS32zZlV25wuWX2OWba8vppnFftsp8+rl93pzw/XyuX6WNFyfHvGtqqIptkGcLbj65hbKoIxcTyS8V7J9cH96/Dl+cWSPU3orUHNz3p8eZZ/uF7eX7JNz/JC2bZSNH5Gjc9MYTfiK1YnyZRyW3Q/YGRwR/TdAEpKo7AcvobdMlQWUeSE6VftE4THOJo58P0FCkc7gDsAjR58jZyoVK1Aca5zwLawqGjw5iY+QntbEx+m3x48H9zQRNOCE8vUZhfJfZr2Wg6eieBeDjEf5j0aXidwmBzgpRNfQ67jB+bGeD8Q3d8YXI+FPKCiwGZd+MpbgYI86zjPbodqBC9j56Lpmxw5GnTaebjy9gwSjAl5KZkL9bxbFfBM/CZvHa+ZJaLL3uiZEV05oHMD31wOPgI/2iKLEceteIAWD8/7ZDEcymc6xH1kdilZkZQMDRq+RSBXH2cs1Fe7QqxB+dt4MT1kViqlOiOfKG4/xOEL5h1aP+RyKwwNxufKJh40uKWJuwUnzcPtAO7l8BiXB2WyMTEbFJADNaeAJDTXSugwOuHkpY2SfJMGviX6ju3UyDnrKPm6Q34bftLMS8vLX+hCbF6COtsEZCM+4Ye4mPucekjulxGji7WCHEmP2yzRwZ5V0KkM/mATzBx3Uh8TNT/4+5pZywlKRuTaYvvS9Z6La/jQRP7w1CfHDo6S53E1sZvj75S/nYyrg5AfGr6e508nQj5FutSJX57Mqx3HIvhjKd5nbDgxMd5sT+LtIou9LPIuqalDhaBLnnZLCjUvqf1IvTGLpF+i6ZL7RyfG4X1SB0ZKVjnq3Zges0xmD1r+RcMjAB69xvwJT5A6Jqu2E9UBeuwaMBb37hscaz5obX1rRcWt/kfXISbWiyyNrPyQ+EPAG0KSntOsznpI1gdXTWfWIry29Lxt0X8U3+8cBfAGjrw0vTidXu0+RMNHBD6QtEYaEj1CvdH2vtp1xeRLag4Sp7ekNXWIF2dkmiCOMyYupl0mfyvN5Ty3itcotlBjYLyKcu6sRI9915idSV4N7OxFi1VJ4oMXL3H22AZgW5DTQp+rObx5r8wuMO6gXNeSTUhuL7hWtRDm9iR905BCHHXjCy/79PtBNie3hbrW6TMq15juSb5+wMKZqWXcfiSes5B+DvfvYwen8LO4+UonwCuar9DjhgU2gTa4UWAvVxJHG1B8zxC3BgLHwbgmusk71qzpY4eOfa/O4S3NOjC35xoq4JUC7loQr4bQ75O64dcrFs/mQUdqzZKVdq1endEX5UvQX65kPM1rvl9JWFO4/cEUASX1wvPLfrh+HTcu9L+V3ZNYn5b5VS/Pr4rh3kYDRye3DhVMzwplEeXZEQEvXxI8e1wQN7K5ClMXsN8dGD+0f4rlF+Zymo5KDtoiiZV7BLWL1Maq5deqDsMffm99E2x59mRC3arKIew1Z6pmgSNrG2r97KN4jsuNXxXQIj5WdWsOZ94KdbsE4K8lpKmTf8laUMF15qyqn/ddKY+nFHOn6N0r3X+kyZdMTqkcC9pk6T5l5z4J7u9wnvP2KGH9l+GM623g3PikhJ+phLXhPglPn5U8z18DPkDDOusUNPw5yXPeHu7Vphc6NkhPMEy+Cn3WB/BcCrqivQvRu1slMI8WPPvAzAWpPRf63XtTyEXFq9Z3Gu8ggM/yZBiyi401Q2Z/HoW5o3EGpU2iE7x3tzHUyd13jzkztmP7dYUacS/irHVReOix388gBpi5RNGemUHx8z6mD54hoLAmsmc0QhpxOrmdU7NFcn9GoyYPAPjHVzjv6MInAbxOXpuN/0r8gMSE7S1YVbYfyqJOP69Rp58X2LabY1umP6fkiustO6lnkJ9umCNy/HHYR+n5/PYmzyvnD3LUvSieVujy1wwrpVq0Zhh3VikcV66V/NZxsC8nfBRcjI29fzw/QL/bAWR7WVCDzsloerYTQ3M3TRPa9mXBM0iTfvYKn9YuJJBBRouZ5x/P9+eLRXK+cGX+tLy8vBj8ezS4OvABlJ9Tn18El+TcF6RDcu0sAWNlfZUvaz/9DrTlORSfq8N9vIo7Hx1g5eC+AwF890tsQcOvA/iiiv5Qa7zI/BDqiYb/kNAXeDSYtRziCy7ZN0/ryzT8pmDsGxz9xdmCx7vIFm8BWzyIIlt0IfYT+TL9/msKeoti6I5GDIlkelviy1B3Mhkhbhq+zIGT+FuWuYuGf5eRT0E9vKOh0/MSe11W4Ov3EvniYjZJDEG7J9GjLGZgH7Usyl9nRi8sBH+bg78zi5vP4FNUsvwFdUPBBvAVfEg/ebwmoJ22NkJ/TawPUA9V89V5jj7S+jT04XcEuHX1kzZWePIn1Z2qvN2KMZG2ltLwnwH8N0EdkOG6IMn7Mr0nrb/QJveL6wvRKzc+guYfPf7G0pHrx/7Zb7772DcKI+ufTRAfij3wXiSIkRQ98ACnfkt9R7GX3YME+FRiT8dPOT3fLpWeT+avIP7QsqJORXkR6lnU48h0+EcO3yp8ZaGrvwL4Hxq6+pckL14W4FbpbXj+xomnXY14UtHFavSHFzVqC8y1Ov0htM9bEr44cbo7y7kZ7MlEZ7IlvaNxg0JcquZ+ms52Sc7n+OFuVT+E/cNOjZiEOQbONxT8x7gtI7tDHmTrOCLd8PJx0rob+fSeDGuPsUOSp+J8SXH+AmuaUh6AsQPnQgr+ZXw0G58geFLmAqJzWS6g+8Q5RM2jHr70idM3fPrgv1997olNhVMvfVdtHmVsk9g7zboFXF/7jXrO2aOac2Au/nCG/jWgoM87M8oxkId2DV3o1hZOzhnIMud8KkM8NDyuUXd+C96dFOtQGXfCHNsSO0lyN/SZtLUS5jPoQ7yzBEl9Wya/Su6m4Xs05IW6G1V4d2yVasi4Bv+TcTUDJ9hzuaecXz+8a+yuc2d3dlx6aU5jbQHkeuNWAE+p8IGU1kQNcGbHgGsP96nntb0Zzg+ktRXqTSV+0voJzJGTivrOIk+D390Y4OyYUv8GfeCYOE8R3DR8QoHWI9TY6zT84lYQE/jn2ysxsXBw4bW2oSM/+PZMz9lNxhcnkdo+Ac83aPiUpp1ovusNvgOlohdfeW/7zu7Jww9efOCX5/9y19tqfHPtmJiWYs/LiwGoIxoWnSXX2fcTyV/UsBOIgZZ4ytJv8Q9HV9arLy33vtk7//HOZxZ7vr7wpx58diBLvz2t4UswvzyRoW5VcMn87jRS2A9AavGVtMdO0qM0xnZp4BkEsGhPLWmMaa5BKO9z0e9K1tWNLg1asvW0juR6Z/as31PgQ7IWZ4jOXcrmqFuT80HW8Wh4RKAPlfUu+PtHjbMAcP1BhSdGNwMa8t0J4H3pbWZ8E8A9CjLBNdN3OfGSdn/skiT2YM8nq+f02MWM8iasSQ9p1KBHwPitSGF9ELXWjXWKMnHW6vby9n1lcy8oX1Zr1zT8bPqcy8zFz0h8TMWn6HmE6tlakV/APifLnkln3gB7JhVcsnmBsAdlzyUaTyvSXo11yZvT+yXTJ39P4pcq8kK7wfPMK7rGeeX1kf/9femmJ/9zYfvlpW/d9JGi4hwM2hWuEwlpIbXedxHAjwL4RQVcZjb1gLGjynwP+hNvvkfDz2ngrqbHxcgIfuuoVCMeAvBTAj9XrWk0nh8CWGV9CMbPTzVqxFcA/BPNPEbDP9LgC8o4BeAXNPiCPYQKLvB7UeNXAK5lGAMquKDffjm9HaXxpOKrMCee5eRE5nd7O/JHMU3mN4MHxveP/h+amWuB", 2)'
  I_C_1 = [0.00455  0  0; 0  0.00454  1e-05; 0  -1e-05  0.00029]
  I_C_2 = [0.00032  0  0; 0  0.0001  0; 0  0  0.00042]
  I_C_3 = [0.00223  -5e-05  7e-05; 5e-05  0.00219  7e-05; -7e-05  -7e-05  0.00073]
  I_C_4 = [0.03844  0.00088  -0.00112; -0.00088  0.01144  -0.00111; 0.00112  0.00111  0.04988]
  I_C_5 = [0.00277  -1e-05  1e-05; 1e-05  0.00284  0; -1e-05  0  0.00012]
  I_C_6 = [0.0005  -5e-05  -3e-05; 5e-05  0.00281  -4e-05; 3e-05  4e-05  0.00232]
  I_C_7 = [0.00795  0.00022  -0.00029; -0.00022  0.01089  -0.00029; 0.00029  0.00029  0.00294]
  N1 = sym
  N1.s = 'symobj::fromString("eJzVGktvG0V4/Aip82pArUIhVV0KXHqBSoDUqsWJ81CkuEE0VFElWDbesbuwD2d3ncQVhyAhBAiJC/Q/9IoqbpxAlUAc6Y/gD6BKRDI7s+t4/M3szPrRKLE08n4zs99rvtfMbA4hlEXo4GH4n89lxsK/0iso+uXC53PxczgHFUjzW77u+2bdod0949dI28OmZxR3dc/Uty1cdHQb+8Wmj42i6RT9lu1uf7bUtO3WmoGdwKyZ2EMszSzAmSftvmsZYE4Sj3S+b7kB6H+BND8wLHOb0ptA3d80aT4O7rTsBcvUfexHsl1gaPzJzB+Zws6TlqiTdEp5Pe4PGSldiZ8zQEmDKCxH2pJrQ2VRRVb0wDP3KY9JNHPg+Q8GRx7AY4DGWdKW9xseDhXnOismJqKi0qtdfJT2pS4+Qj8fjpdmumh6cBKZsqZB+1nakwI8lbAvh7gf9x4LT0kMJgd4GSet7DpBuNwE7+W4fzZs30Q8IEOyZmdI03CoIB/viNZto0nxcuts6IEukKNDJy/CpZk1JJkT8WLpD1qa60l4pnaj4Z2mblFdzsdjmbjlgM4zpLMd/iR2NKfyEcdt+ICWCM/LKh+O5NMdaj6qdbFwLCVHg4UvSuQqCuZCfeX78DUof1bk02W90bBanHwyv31TwBeMO6x+aHMbHA3O5mydTCrNdXH34GR5uArgeQGPSXFQJRvns2ECWWk6VaSgOamgw+lEEJdmFfFmEPhi/EzWqRNzphj5ChG/HTvpxqV2+8sziI9LUGcvAtmoTQQRLq5fkA9pv404XUxKYiQ775xCB+88B52q4De64Mhxp7UxWfFDnifq2AlTRmza8vVl870Q19JGRbuz+eHa7VU6npQTCwJ7Z+ztICkPQn5Y+CWRPe1HfMp0OYz/imR+3n4sgxcHeJ9bw0plvVueJK+LyvdGEXdpTi1Xwyp527X6yHlp14/mG92g9RJLl/ZvVdZhP80Dyxa249qNqzFtunsYyr5YeBnAq6fMnsgGaewDz3TiPMDOnQBzSe0+4+C9sLQN8JGKe+2PzUOcrxs8jVHZIbWHkDeEFDWn7tV9pKqDPd2pY8prT82bjf9Rcr2zBeAZgbwsvSSdnnQbYuG7EhtImyMzCj1CvbHrfdJ1xcVLZg+SpLe0ObUs8jO6TZD7GecX2y4Xv/vay/muR84o5pg50F9lMbeu0GPxlK0zjavhOvvxYVUa/xD5S9J6XAKwKYlpkc01HdG+V7Uu0O+gXKdpTWhsr7rYq0axPU3dVO7DjwqkkWOfa0EYzWm3VNfD1BmNU6Z7Gq8/xyQy9cxbQPI9C63nSP2+dnuTjCXtV8YBXtl+hZ23JFkTuAbnJevlKvxoBiXXDElnIHAe9GuqG83BdT0gBp34XkvA2yDnwMKaq1wlJwXCsyBRDmHfp3kjaDWwaM3DihTX6Un7ULU6py/GlqC9HKc/7Q35fiNlThHWB5sUVOQLP7CD6Pw6aV5kf0e3J4k2rbKreZFdGdHdRgfHuDAPVXUfR7LI4uyyhJdvJWPfSfxGtVfh8gKxu5X1jYVNnl8Yy1k6/cSgOYWv3JTkLpobPRw0PYfjj7w33QV7xn5Iqdt+5ZDWmjVPrwpkzaLe3w2G56TY+KOEFrUxz206gn0r1O1DAP+UkuYw8ZeeBVVdZxd7gRa4Sh6/7jN2yt497vpjkHjJxZTG/bBMVt5Tjt9Q4H4kGBfdUcL8r8KZVNvAvfGBgp/NlLnhIwVPnyjGtVNgAyw8zDkFC3+qGBfd4Z40vbC+QWuCJfootdkAwLsD0JXdXcjevaCARbTgtw/cXpC5c2HfvTWAXIy/DvXM4i0B+LFIhrJpdM4Muft5FMWOzjcoWYVOyN3dbKST69fXnJrpmEGrjxxxCwnOuhg87NxfRuAD3F7CMGs1lLzv4+rgGgWlOZH/RiOikaSTq4KcLZP74yFy8rsA/vWY486w8AGAp9S5OXOosAPqE6b/AHt8PTSKPP1kiDz9RLK2BcHacvU5I1dSbTnOjEF+CjBG5MTziI2y+/nXujwffX+QY/pif0r0m2ivZjctwbcGNEbsaG9rhkG/cTuq4dvtdrj3RF+RdwtEsMWfDw7/+35y/68Sfv/Rv/8IaLIy/A3gpwC31cFNjGfn93tfvLW4//i36WeHN59efi8Fbvn9UcPdiz+c5O4sQlkRwHevH97ib664uHRF29JEMXFlfWH1f/RMSo4=", 2)'
  N2 = sym
  N2.s = 'symobj::fromString("eJzVGs1vFFX8dXdraYFaCKQiJSwiXrhIg2j4Ssu2JTUtGKimAXWc7rxdBmZntjOztEs0qYkaNUYTo/wP3ok3ThgSPXCiJpJgevBgiGfjoUmd92a2+/b3vvYLQjd52fm9r9/3x3szaYRQCqGV29F/Jt3TG/2NvYziXzp63pM8R3NQP2lBNTCDwC66tLthfJS0JWz7Vvam6dvmgoOzrlnCQbYSYCtru9mgWvIWrk9USqXqtIXd0C7Y2EcszhTYM0PaNc+xwBwZjXR+4Hgh6H+BtCC0HHuB4htA9d9O0gIcXq6Wxh3bDHAQ87aPwfEbM79rAttLmlQmzQnl1aQ/ImTscPLcA4TUjsDSpE14JSgsKshZM/TtZUqjDGcaPP/K7JEBcC/A8SJpk8tlH0eC89wpGxNW0dj++n4U98H6fgR/JhofG6xv07An4SllW7Sfxb1dsM9s1JdG3I9bx8I7FAaTBrT0kZbz3DBSN9n3UNI/FLUvYxqQpdDZNtIMHAkowIsivV2s0H05PVtmaAr4qOHJiPYy7AJSzIlpccxbVcPzFTRTuzHwYsV0qCxHkrGepKWBzHtI50b0U9jRsM5HXK8cAFyifV7S+XDMn+lS89HpxcEJlxwOFj6g4CsrmAvllWnB1yD/KZFP58xy2aly/Kn89jUBXTDusPKhzStzODibK5lk0thwfe+GPVkajgJ4RECjLA7qeON8NkogUxU3jzQ4t2vwcDIRxKUhTbxpBz6QPBM91WLODoa//pjemp3U49LGxqfbEB+XoMx2Ad6oTYTxXly/IB/S/hLiZLFdESPZeXs0MnjjKchUBx+pg13fu1kbUxU/5HmgiN0oZSSmrdYvm++Fe01cnDUuz12avnCejstyYr/A3hl7W5HlQUgPC+8W2dNyTKdKlp34r4jnp+3HKvhcG+s5Hc7OztTLE7ledL7XjbhLc2ouH1XJC57TQs5rVn8035gWrZdYvLR/fnYG9tM8MOngUlK7cTVmiZ4eOrIvFp4E8PktZk/kgNT7jm+7SR5g5w6AuaR2H3TxUlTahnhTxI32x+YhztctHke37JDaQ0QbQpqa0/SLAdLVwb7pFjGltaHmTSX/SF7vzAN4UMAvi08m0+fdhlj4PYUNNJsjezRyhHJj9f28y4qLl8wZRCa3ZnNqTuRn9Jig9jPOLxY8Ln63dJYLPJ/cUQwzc6C/qmJuUSPH7BbTM42rkZ6D5LKqGf8Q+YtMHwcBbCtiWmxzFVd07tXpBfod5Gsr6YTG9ryH/Xwc25upm3It+FE/aeTaZzSMojntVsq6kzqjvMVkT+P1DUwiU8O8caQ+s9B6jtTv0xfmyJjsvNIH9lWdV9h5EwqdQB3sVejL0/jRIJLXDLI7EDgP+jWVjeHiohkSg5auqwpoa+ceWFhz5fLkpkB4FyTKIex6mjfCahmLdB5VpLhIb9o7qtU5eTG2BO3lWfrTUofry03mFGF9MEdBTb4IwlIY31/L5sX2t/n2RGrTOrsaEdmVFb/bqO3RJ8xDeTPAMS+qODupoOUrxdjXCr/RnVW4vEDsbmrm4vgcTy+M5SyeVmLQsMZXzihyF82NPg4rvsvRR9btrIMNY981KdtW+VDWmgXfzAt4TaHG3ymGZlls/EGBi9qY71VcwbkVyvY2gH9sEmcn8ZfeBeU99yb2QyP0tDR+0WLsVK191vVHO/GSiynla1GZrH1P2XdKs/dPgnHRO0qY/3V7ymobeDZe0dAz12RueFdD04eacWML2AALd3JPwcIfacZF73CfN7mwvkFrggn6qLTZEMA328CrenehWrtPA4twwW8fuLMg886FXXu2Db4Yf+3omd13DMB3RDzkbKt2Z8i9n0dx7Kh9g5LSyIS8uxuKZXLy5LRbsF07rLaQI84iwV0Xsw879+cu+AB3lrDsQgHJz31cHVygoDIn8t9oxDhkMjkqyNkqvj/oICefAPDdZxx3OoVXALxDn5t71jV2QH3CDm5hn6+HupGn73eQp+8rdNsv0C1XnzN8yWrLPmYM0tMPY0RaPI/YKHuef6VO8+b3B2mmL/Enqd/EZ7WyU0nuDNXzShVH8E0CjSWLxqhhWfRbuM1af2NjIzqjos/IWnJIWT305r213x+fHvq+d2at+P5bgLZewOuqgp74XVDZW0o+guTePywaxxDY7wqSnyfomrwXSPYaRbq1gc2dsx8DWZRrsiAvlkYerF9PXz0y/8/u1avHP39wA3yvBePJQ8XYKhKc/ak+vBAhuV0/VIytCnhh4TUNPSz8CMB/CvZi5US8aNNmvq0s7r976fah47tOnP7m7ScZjZygLBLbPFazTUhH03iR3lZVPIvkx8J/d6B7Fv6rS/p+pJj7h4aXKy3QC+UCdfIJSnSyDfG/xBaE8YYknsVfrnz8+rnlO/d2/rd+Jgo+TdgOCz/R2KkSF+quvUCf+RcJ6p/DxryBBLXX1Mz4+f8BjpbQ+A==", 2)'
  N3 = sym
  N3.s = 'symobj::fromString("eJzVG11sFEV4rneltLRIFVIRCAeoicKDFCQBhLT2h9S0YKAaNOq5vduWlbvd6+4e7ZEQa2IMEqMvgokvvhk1vmiMbyT6QqIv+iASBMJfMEgkBpWoCVp3Zvd6c9/Mzuz0FkIvmXS/3Znv/29mt0mEUANCU8e8v6lkotH70/UA8n9J73pxcO3NQc14OGVHcxxjzCS3a5534jGhG3YufUCzDW0kr6dNraA76ZKj59KGmXbKBWvkld5SoVAeyOmma4wauo1omg0AZwqPfVY+B+aE8UjmO3nLBffn4eG4ubwxQui1oOqvDQ9Hd/eUC915Q3N0x5dtKUXjW2p+bApbgkeoTqIp5cHgvsdI15rgOgGUNBuFJfHotQpQWUSRQ5prG5OExzCaSXD9DYUjBeBGQOMePPomi7buKc4y+w0di4q6llXxEdorq/gw/ZT3vGthFU0NTixTg5Ej92naCzh4hrx7ScT8mHU03CpwmCTgpQmPHst0PXNjvKuC+4u8cdjnAeUENpuPR0b3FOTo4zy77SoRvIydc5qrceSo0EnxcGWMUSSY4/OS1w6WM5Yt4Jn4TUYfL2l5osvlwbNEMJJA5wl8c9r7CfyoQxYjplV0AC0envtlMezLp5nEfWR2yeuBlAwNGl4hkCvNmQv1lVKINSh/Ay+me7RiMV9m5BPF7cMcvmDeofVDhlVkaDA+V9DwpK6OKu4anDQPawG8nMNjWB6UycbErFdA+ktmFkloLpDQYXTCyUuLJPlmNvCK4BrbqZJzWin5mn1+K35SzUvT06/NR2xegjprB7IRn3B9XMx9Tj0k9wuI0cUCQY6k5y2W6ODx26BTGfxQFYwdd1QfEzU/+LplTDe9khG4tti+dL3n4urdNZTZM7x7YOcO8jysJjZz/J3yt6mwOgj5oeF7ef406fMp0mU98cuT+XbHsQh+chbrGRsODQ1W25Nwu8hiL468S2pqT9brkkesvELNi2o/Um+0HOmXaLrk/t6hQXif1IG+vF4IejemxyyQ3UNd/kXDfQDeMcf8CW+QGp+2DTOoA/TcFjAX9+4LTX3Ca21dfUbFtf5H1yEm1nMsjbj8kPiDxxtCkp5Ts8ccJOuDbc0c0wmvNT1vQ/AXhfc7ewG8kCMvTS9Mp3e7D9HwswIfiFojExI9Qr3R9r7bdcXkS2oPEqa3qDW1hxdnZJsgjjMmLkYsJn8r7eUcy8ZnFB3UHBivopw7JtFjeo7ZmeRVz85OcFgVJT548RJmj5UANgQ5zfe5ksnb98rsAuMOyjWXbEJye9bS7ayf26P0TT0KcdSMBz726XS9bE5uC3VdT59RnGO6J/l6v44zU828biTes5B+DvfvAzuH8bOw/UoTwCvar9DzegU2gTZYIrCXJYmjhSi8Zwg7A4HzYFwT3WRMfUxzsUOHritzeJvNOTC35+rJ4pMC7lkQr4bQ60ndcMtFnWdzryPVx8hJe129OqMvypegv9zJeJqoc30xYk3h9gfDBJTUC8ctuP75ddg83/9m3p6E+rTMr5bz/Crnv9uo4Gji1qGs5ui+LKI82yfg5U3BsyOCuJHtVZi6gP2uf3BX9zDLL8zlNB2VHNQhiZVtgtpFaqOtuyXbZPjD69qqYM2zdyLqVlUOYa85amtZjqwNqPa3leI5LDe+K6BFfMy2SiZn3wp1ewzARyPSrCf/krOgrGUe0G0341pSHt9QzJ2itXe6/5hNvmRySnGf1yZL31M2bZXg/pjznPeOEtZ/Gc6w3gbujack/AxHrA3PSHh6SfI8Mwd8gIbrOaeg4Zclz3nvcO82vdCxQXqCXnIp9FkXwAdmQVf07kK0dqkE5tGC3z4we0HqnQu9dvss5KLita5rGm8XgL/gydBj5Cpnhsz7eeTnjso3KA0SneB3d4t8nWzZMmCOGqbhlhVqxHbEOeui8NBzv4whBpi9RM4YHUXh+z6mDx4loLAmst9o+DTCdLKWU7NFcr9YR03eBODjdzjv1AtPAbhVXpsTtyR+QGLCcA7qNtsPxVGnT9RRp08IbNvMsS3Tn1NyhfWWTdQzyE8zzBFJ/jzso/R+fnWV55nvD5LUvSCeZui2It5erZgvBWeGYfHlzyuU8pxvEkguGc9syORy5Fu4mV5/enoaHxK8jtd6xkLth0/dfHXt6c8+/+3Ihc3vXfoE8AZj6CTi7GkJHcuFvNLrfpDgDNtTEB06hgnlI/c9ulFpwmdQjgAf/uazZt5ZCkdjNBzrkUyerOVAOmcEPvoTgM8Bex5CgT3nI/YXfHMWeT6S25+GL0r0HyYjzx40fF6gjwscfcBeh5YXZwAirxfQ6PL+79Zd2/zLoZbW584dfX/b95Jv8k5K5IsqD+TxooKOzwP4ksBH4bmuCo9nVPSG1PwEynAVwL8r4OLpkubbrPCND2HeLo0vO7772KqN7ZueeOupaylFviGts4CWS+toZfue1R99vbH13/te+PSryXltwLd4+UOko4scu0emDeRUpc3zMRq+qV4jOlVqhGo8XYrRF6GehfUS2FhG+4okVmn4DwD/GWOMzPgOrgFtH2p/f3BhpO/Ehn1X9994BH6nXG+MCOPxNsRImJ/GHAMJqJfLCjER9GfrK/2ZyB9PqePt5OGFulLJubI6HxXPfzHF/3kwl/0mqWhNBP+MI7Lp83X4ObTTZQD/HB13olXCJzy/UbBdAu7RYC5X8QMYA/AdynUFXKdj8gXo11cU1kJdXBPIA22kwuOPAp3L1kKebinqmIZ/FeTHKLFL2x7ug68ryCSrgyo9q0quVOkDVHDx6m1c/a0oXuOul9frwC3rGVVyFoy1OvYLTP4DOkikFGwD14L8l5gXX15WwcXNy5H7PaS2JwI5JbECwI9JciY9N61AF+TBRAun/kbFdQPgerQOXLIc+w+gtQbA6+LzZaV8LvFl9Fd8vqyCS9ZjKMWFzFcxLuadxZrMXvyulnlf0j/YveN/zuV7mw==", 2)'
  N4 = sym
  N4.s = 'symobj::fromString("eJzVG11sFEV4rlco5acgQioCUgUMEaMBqgkQSLEF0oSCSiUFIsf2bnss3O0eu3uUw5DURAz64otggsF335VEE1+MIZEY8EEgCmgEQgRECCE+GJK6M7vXm/tmdmbndiH0kkn32/n5/n9mZptGCDUhNHLc+9ucTk3w/nQ9i/xf2nueFTx7Y1Arbk7F0RzHyJvkdV3/ctyGdcPOdRzQbEMbLOgdplbUnY6yo+c6DLPDqRStwb095WKx0pvTTdcYMnQb0TibwJrNuO2xCjkwJoxGMt4pWC54PxE3x80VjEGCbzKq/abh5uju1kpxXcHQHN3xeZtD4ThDjU9MYLNxC5VJNKEsCt57hHQtDJ5TQEiNCCyNW49VhMIiguzTXNs4SGgMw5kGzz9SazQDeALAMR239QdLtu4JzjI3GDpmFXXNra1HcC+orYfxN3v9XW21ZerWxDw1GTnynsY9hbNOn/cujZgfM4+GpwoMJg1oacGt2zJdT9143eeD9zO8dtSnAeUEOpuEW0b3BOTo+3l621Im6zJ6zmmuxuGjiqeZt1bGGEKCMT4tBe1QJWPZApqJ3WT0/WWtQGQ5L+hLBS0NZJ7CL0e9n8CO2mU+YlolB+DirfOMzId9/jSTmI9MLwU94JLBQcPzBXx1cMZCeTUr+Brkv4nn091aqVSoMPyJ/PZFDl0w7tDyIc0qMTgYmytqeFBXe23tujVpGpYCeB6HxrA4KOON8VkvgWwom1kkwTlFgoeRCScuzZDEm0bg+cEz1lM15kyl+Gv16a3aSS0ujY6+PwmxcQnK7CnAG7EJ11+Lec/Jh+R9ETGymCKIkfS4WRIZvPYIZCqDF9fAxNeOamOi4gc/T87rppcyAtMW65fO99y1erb0Zbb2v927eSPpD8uJrRx7p+xtJCwPQnpoeCbPng76dIpkGcd/eTw/aj8WwW80MJ/RYV/fplp5Eq4Xme8lEXdJTu3OelXyoFVQyHlR9UfyjZYj9RKNl7wf6NsE35M8sL6gF4Pajakxi2T3EMu+aHg9gDeOM3vCG6QJb9qGGeQBeuxkMBbX7m2mPuyVtq4+JuJ6+6PzEOPrORZHUnZI7MGjDSFJzanZeQfJ6mBbM/M6obWu5m0K/qLwemcAwG0cfml8YTJ90m2IhrcJbCBqjkxJ5AjlRuv7SZcVEy+pPUiY3KLm1G6en5FtgtjPGL8YtJj4rbSXcywbn1G0U2Ogv4pibl4ix45xpmcSVz09O8FhVRT/4PlLmD4WANgQxDTf5somb98r0wv0O8jXeNIJie1ZS7ezfmyPUjd1K/hRK2742Ge560Vz8loo6zh1RmmcyZ7E6306jkx149Yh8Z6F1HO4fu/d3I/7wvYrLWBd0X6FHtcj0AnUwWyBviyJH7Wh8Joh7AwEjoN+TWSTMfW85mKDDp1X4dDWyDkwt+bqzuKTAu5ZEC+H0PNJ3nArJZ2nc68i1fPkpD1Wrc7Ii7IlaC+P05+GY84vRcwp3Pqgn4CSfOG4Rdc/vw4b59vf2O1JqE3L7Goez65y/t1GdY0Wbh7Kao7u8yKKs+sFtHwk6PtY4DeyvQqTF7Ddbdi0ZV0/Sy+M5TQelRjULvGVNYLcRXKjrbtl22Tow/Om1cC6vk8iylaVD2GtOWRrWQ6vTaj+t5qiOSw2firARWzMtsomZ98KZXscwMci4owTf8lZUNYyD+i2m3EtKY0fKsZO0dzHXX80Ei+ZmFLa45XJ0nvKltWStb/k9PPuKGH+l60ZVtvAvfGIhJ7+iLnhHQlNuyT9mXFgAzQc55yChndL+nl3uE+aXGjfIDVBD3kU2qwL4AMN4BXdXYjmzpHAPFzw2wdmL0jdudBz1zbAF+WvsZ7pdbsA/BWPh24jVz0zZO7nkR87qt+gNElkgu/uZvgyWbWq1xwyTMOtKOSItYhz1kWtQ489lYAPMHuJnDE0hML3fUwdPERAYU5kv9HwcYTJZCknZ4v4fjdGTn4dwN895rgTFx4B8FR5bk49lNgB8QnDOaTbbD2URJ4+HSNPnxbotpWjW6Y+p/gKqy1bqD5ITyuMEWn+OGyj9H7+hRrNY98fpKl3gT+N4Z2GeHu1UqEcnBmG+Zc/rlgucL5JILFkf6Yzk8uRb+HGav3R0VF8hfwBnos/lvjm6N0fPrePDH8/c/qSopM9BGiDPnReoJNfBH3nUfi+gcgpazmQB/Le4wHKQAUnZ73lSEaLY5ghtKyg506Ihm8ZxEfP+RXAvwvGXgHwZaDXwyjQ6yTE/iTfnkH9iPD+JtFHGD88nDT8p4KcLlNjJynaBOSFliE2QiJDz/nRjlMX2od6R07cnZt57/a2c71AhjzfoOFLAL4BcNlVXPhSc97Zh3vTOxcP/D3z/M7OI2f3Ibkf0vBfElwHqri8AI2G83dO3d/+RcvuBSe/XfXTZ+2KuC4D+KqKDBVxQRneVuFLUV9QhrcBfE/i+9CWafgagP8A8AMAX08gBse1GWE8QfH1CPcnj9yfr+079/KtlTcPT566/cqxE2t+jskDlNdYXsW4Lr3SefG5yye/vnUmX9k1cthVxCXTjTB2KNq9kj9DGcaMiSIfi+mvKfrMOWF/TU0E/Q8VZRA2Fts6p45bUa3jRDiYuwav1smQaY3XTyI7uabAM5TvTYm8r0vo4shoWVVGIjz/NG5fqdkcG0hK54p6XaGiVxltMBfdiGHbVyPE+bC4H2XtBPhNtUVcR6Ve5X8XV7KGg38IE9n6jhixGtr39cZ1l3paQifU3UOJrDg+upzno7zYqugPnUnGOZhX7ijMjernUeoYlXgoy+eNxmlZHkQx4ukS0P9AwVbhOSGsWYRnHIo1C+R5Eei/qED3SwnZKKyj7sTQw6uSGKKiF/i/Z43yB/PIDYW5MJ/BHETra1oMGi8AWKW2APqDtQX6N4Y+4VoqNTWkC/rovejygXaVEt1n8fyEhpcBuDmGfCBP92PGnQZ9RRpXFOyJkdfKxnmsiyVx9+I0TZ2N2yGsSePkHaa+VfFbXm5tMBdI98IqtiTbCyNqraTPri5y8odKvqDhNQLdJBirlfZuo2DuW6BfZQ8jifux4hpeK/J5VLxzGxhDUwMJxvamGDJIMF+h/5LLC0rxSpIXVGxXmhcUagOZrxK6mPv/hZkB/N0T8+3Bhk3rNv4PPC82Ww==", 2)'
  N5 = sym
  N5.s = 'symobj::fromString("eJzVG11sFEV4ttfaH0pFA0GwSBEkGh6UUiCWnxT6Q5q0YKBqQ6Ln9m5bVu92j9092kNNMDEGfQBNlBcfjNHE6JuGGKMxPmhI9NGAREFAghCiIYZIYgyx7szu9abfzM7s3B6EXjLpfrsz3//fzG5TCKE6hA4d8//Wp7QG/0/PUhT8Uv71wvDan4Oa8XBLru665oRFbs963onHpGE62Y4DumPqYzmjw9LzhttRdI1sh2l1uKW8PfZ8XzGfLw1mDcszx03DQTTNOoCzHo99di4L5kTxSOa7OdsD9+/Cw/WyOXOM0GtBld98PFzD21PKb8uZumu4gWxLKBo/UPNrprBFeETqJJ5SVoX3fUZ6VobXGlBSNQpL4dFn56GyiCKHdc8xpwiPUTRT4Pp7Ckc9gBsAjbvx6J8qOIavONsaMA0sKuq5v4KP0F5ewYfp1/vPe9oqaGbhxDLVmVlyn6Y9j4Nn2L+XQsyPWUfDrQKHSQFeGvHotS3PNzfGuyK8v8AfhwMeUFZgsyY80oavINfYz7PbriLBy9g5q3s6R44ynXoerrQ5jgRzAl5y+sFS2nYEPBO/SRv7i3qO6LI9fKaFIwV0ruGb0/5P4EeLZTFi2QUX0OLhuU8Ww4F8ukXcR2aXnBFKydCg4WUCuTo4c6G+6hViDcpfx4vpXr1QyJUY+URxu5rDF8w7tH7IsAsMDcbn8jqe1LO4gnsWTpqHNQBu5/AYlQdlsjEx6xeQgaKVQRKa8yR0GJ1w8tICSb6pBl4WXmM7lXNOKyVfc8Bv2U8qeWl6+pUmxOYlqLN7gGzEJ7wAF3OfUw/J/TxidDFPkCPpeQslOlh/C3Qqgx+qgDXHHdfHRM0Pvm6ZMCy/ZISuLbYvXe+5uPp2Daf3jOwe3LmDPI+qic0cf6f87VBUHYT80PC9PH+aCvgU6TJJ/PJkvtVxLIK3V7GeseHw8FClPYm2iyz2apF3SU3tzfhd8pidU6h5ce1H6o2eJf0STZfcHx0egvdJHejPGfmwd2N6zDzZPSTyLxruB/COOeZPeIPU8IRjWmEdoOe2gLm4d2+zjEm/tfWMGRXP9j+6DjGxnmVp1MoPiT/4vCEk6Tl1Z8JFsj7Y0a0Jg/A6q+etC/+i6H5nFMBtHHlpelE6vdN9iIafEvhA3BqpSfQI9Ubb+07XFZMvqT1IlN7i1tReXpyRbYI4zpi4GLOZ/K20l3NtB59RLKbmwHgV5dwJiR475pidSV717eyGh1Vx4oMXL1H2WA5gU5DTAp8rWrx9r8wuMO6gXHPJJiS3Z2zDyQS5PU7f1KsQR8144GOfTs/P5uS2UNdJ+ozCHNM9ydcvGDgzzZq3DYn3LKSfw/374M4R/Cxqv9II8Ir2K/S8PoFNoA0WCexlS+KoDUX3DFFnIHAejGuim7RlTOgedujIdSUOb9WcA3N7rt4MPingngXxagi9ntQNr1QweDb3O1Jjgpy0J+rVGX1RvgT95XbG02TC9YWYNYXbH4wQUFIvXC/vBefXUfMC/5t5exLp0zK/auf5VTZ4t1HG0citQxndNQJZRHm2X8DL64JnbwjiRrZXYeoC9ruBoV3bRlh+YS6n6ajkoMWSWNkiqF2kNjqGV3Qshj+8bn4FnPXsaEzdqsoh7DXHHT3DkbUOzf5toniOyo1vC2gRH3PsosXZt0LdHgPwOzFpJsm/5CwoY1sHDMdLe7aUx9cUc6do7e3uP6rJl0xOKezz22Tpe8rGTRLcH3Oe895RwvovwxnV28C98SEJPyMxa8OTEp6elTxPzwEfoOEk5xQ0/JzkOe8d7p2mFzo2SE/QRy6FPusB+EAVdEXvLkRrl0hgHi347QOzF6TeudBrt1YhFxWvia5pvD0APs6TodfMls8MmffzKMgd5W9Q6iQ6we/uFgQ66e4etMZNy/RKCjViK+KcdVF46Lmf1yAGmL1E1hwfR9H7PqYPHiegsCay32gENKJ0soZTs0VyP5OgJm8A8Ne3Oe8khQ8BuFVem7WbEj8gMWG6Bw2H7YdqUadPJKjTJwS2bebYlunPKbmiestG6hnkpxnmiBR/HvZRej//YIXnme8PUtS9MJ5m6LYg3l6tkCuGZ4ZR8RXMyxdznG8SSC7Zn16fzmbJt3Azvf709DTWyKt4Lf4w7ZPVh78czBw/8uFC78Uz33z2I+ANxtApxNnTEjq2B3ml150UPDuFovcURIcZ24Xykfs+XSTg9SSAz0jkEvLgmlYED11J5Obg60Qo2l9/5a9ZR69piEdnrYjOLwD+TcITDV8A/vYyCv2tCbG/8Js4ev0VBV8R8XxOYpco+Xg0afiSAg8XqpQF6vSMRJa4vJ+tEZ4/AHxVYe15AF9TWHtdEu9x8ZxT9DloUxr+XZJXoO/Q8GUAXwSxg78uJbGDi/b+7/a+9Nj2qePfzv/n5pZTKzaC70lltM/WSHfnJXg4dWhduQ4p1pXOpHVFZLfLCez2p8SOMn/i6GhtWUeQjkpMxrFvTN2vU9G9TH8XOfkido1A8p4ExiPMLzTM2xur4K6BPjTRebiKT18Cc9lvcwr2ZPhPKSJ/3auggwuSWLgCZG1V0At8Lwn5XCLAHTPOOnlxdlE9PrpqmZtgTbyhGPc0/C/HHrFrChK/kzxVI3mvC+SNU8dk8pZxNSXg8QyAVWottOdV4LerEsh7A9gTOyGxp7/5Rkc3HBl9b/lA06XxL7Sv3v2oG6nlTp5dquUb+iXMw6q9i8jmKrigjACXtqZ6GbVm8Py0gr/dpObCPZxKreX5S7U25PlDpO9d+/Tv9y1z/aq+Rz8YffPwI29V0Z9Cu8SmhZL5OfQBFR2BWNfakcJ5i5qOtAdqlH9hbKrkX5jbePmX5nmzol1EMcCp511x9hY0P0vBc9gvXlHgF/S1Gvi/OGl/Qs8VnWWr2BbKc1VhLezTRTkb5jqVHPUzgP+rXX3UViaoDX8BXGsT+MZ1MV/aRkV91WIfBvMelFehV2fyNXzXAHv19VXWwrsSxALs4U4ryCfr4TYDuEsBt6w3Og1wP54gHgYT+B30YYiLjtP5Cez0U4L4l+USlX6Ol0ti99qK/Y4kPyjlLUkfmkSf2u4EuHi9UZSMMh+Buao7Ph+kb6Lhnur50B4G8NO1i80k+xgmNrHfM+/jV6ZH8XdIzLcAA0PbdvwPO/gCrE==", 2)'
  N6 : sym (value not decoded)
  N7 : sym (value not decoded)
  Pc_1 = [-0.00351; 0.0016; -0.03139]
  Pc_2 = [-0.00767; 0.16669; -0.00355]
  Pc_3 = [-0.00225; -0.03492; -0.02652]
  Pc_4 = [0.0002; -0.05268; 0.03818]
  Pc_5 = [5e-05; -0.00237; -0.21134]
  Pc_6 = [0.00049; 0.02019; -0.0275]
  Pc_7 = [-0.03466; -0.02324; 0.07138]
  T_1 = sym
  T_1.s = 'symobj::fromString("eJzVGktvG0V4/AiJkzQE1CoUUtVQ4NITleDQisrBeShS3CAaUC6wbLxjd2Efzu46iSshBQkh4MIF+h+4I25cK8EVgeDEH0EyO7PrePzNa+11o2Slkfebx/ea7zWzLiGEigidPol/y6XCTPxTexklTyl+v5q+x3NQhbSwF5phaLc92j0yfoe0Y2wHVvXIDGzzwMFVz3RxWO2G2KraXjXsuf7BZ+td1+1tW9iL7JaNA8TSLAKcZdIe+Y4F5sh4pPNDx49A/3OkhZHl2AeU3jwaPldIC3H0sOeuObYZ4jCR7TpD43dm/tQUdo00qU6yKeX1tD9mpHYrfS8AJU2isBJp674LlUUV2TCjwD6hPMpolsD7bwyOMoBnAI3nSds46QQ4VpzvbdqYiIpqrwzxUdo3h/gI/XI8XlsaohnBSWQq2hbtZ2kvCPA04r4S4h5uHQsvKgymBHiZJa3ue1G83QTvq2n/cty+SXhAlmLP5kgzcKygEB+K9m23S/Fy+2yZkSmQY0CnLMJl2C2kmJPw4piPe4YfKHimdmPgw67pUF2upmOFtJWAzguksx8/Cjta0fmI53dCQEuE5yWdDyfymR41H92+ODiVkqPBwjcUclUFc6G+ymP4GpS/KPLputnpOD1OPpXfvingC8YdVj+0+R2OBmdzrkkm1VaGuEdwsjzcBvCqgEdZHNTJxvlsnEA2u14TaWguaOhwOhHEpWVNvJkEvpG+k30axJxFRr5Kwu/AToZxqd//cg7xcQnq7AUgG7WJKMHF9QvyIe13EaeLBUWMZOdd1ejg7WegUx38xhCcOu6sNqYqfsj7fBt7ccpITVu9v2y+F+Ja320YD/c+2H6wRcdlObEisHfG3k5leRDyw8IviuzpJOFTpcs8/iuS+Vn7sQp+b4L13B42GjvD8kS+Lzrfm0bcpTm13oyr5APfGSPnZd0/mm9Mi9ZLLF3av9/Ygf00D2w42E1rN67GdOnpIZd9sfAGgLcumT2RA9LM+4HtpXmAnTsP5pLafcnDx3FpG+EzFY/aH5uHOF+3eBrTskNqDzFvCGlqTjNoh0hXBwem18aU15Gat5j+Inm9sw/gJYG8LD2ZTi+6DbHwRwobyJojCxo9Qr2x+33RdcXFS+YMItNb1pxaF/kZPSao/YzziwOfi99jneVCPyB3FCvMHOivqpjb1uixesn2mcbVeJ/D9LIqi3+I/EW2HzcBbCtiWmJzXU907tXtC/Q7KNdl2hMa25s+DppJbM9SN9XH8KMKaeTa504UR3PardR1njqjc8l0T+P155hEppF5a0h9ZqH1HKnftx/skTHZeWUW4FWdV9h564o9gXtwTbFfvsaPlpC8ZpDdgcB50K+pbgwPt82IGLR0XU/A2yT3wMKaq94kNwXCuyBRDmHX07wR9TpYtOdxRYrb9KY9V63O6YuxJWgv5+lPxznXdzLmFGF9sEdBTb4IIzdK7q9l8xL7O/t6IrVpnV2tiuzKSr5tDHDMCvNQ0wxxIosqzm4oePlWMfadwm90ZxUuLxC729zZXdvj+YWxnKUzTgxa0fjKu4rcRXNjgKNu4HH8kXVXhuDI2PcZdTuuHMpasxWYTYGsRTT63GN4lsXGHxS0qI0FftcTnFuhbp8A+MeMNPPEX3oX1PS9IxxERuRrefx6zNipWnve9cck8ZKLKZ1HcZms/U45e0+D+yfBuOgbJcz/Opyy2gaejU81/OxlzA0fanj6RDNuXAIbYOE89xQs/KlmXPQN96LphfUNWhOs01elzUYAPpqArurbhWrtdQ0sogX/+8CdBZlvLuza+xPIxfhrrncWbw3AP4tkqNvW4M6Q+z6Pktgx+A9KUaMT8u1uOdHJ3bvbXsv27Kg3Ro64jwR3XQwedu4vU/AB7ixh2a0Wkp/7uDq4RUFlTuT/o5HQkOnktiBnq+T+OEdOfgfAv55z3MkLnwJ4UZ+bC/9p7ID6hB0+xgFfD00jTz/NkaefKva2Ithbrj5n5JLVlrPMGOSnAmNEWTzvDzQ8zxObe23I85nvDPCksLSGpnVXaNPzIdd/aLwFZeHmNH1y0zjC358iv7xl7BsZeWVx/a3w9+SM6XYdwV3eX4g5b/T7/S/in6/I/DnEP+n/pNj1/wBemf9ZnfGSGb9ALh1+GEv+Fazn4uvmztrW/4AhMiI=", 2)'
  T_1_0 : sym (value not decoded)
  T_2 : sym (value not decoded)
  T_2_1 : sym (value not decoded)
  T_3 : sym (value not decoded)
  T_3_2 : sym (value not decoded)
  T_4 : sym (value not decoded)
  T_4_3 : sym (value not decoded)
  T_5 : sym (value not decoded)
  T_5_4 : sym (value not decoded)
  T_6 : sym (value not decoded)
  T_6_5 : sym (value not decoded)
  T_7 : sym (value not decoded)
  T_7_6 : sym (value not decoded)
  T_8 : sym (value not decoded)
  T_8_7 = [1  0  0  0; 0  1  0  0; 0  0  1  0; 0  0  0  1]
  V_0 = [0; 0; 0]
  V_0_dot : sym (value not decoded)
  V_1 : sym (value not decoded)
  V_1_dot : sym (value not decoded)
  V_2 : sym (value not decoded)
  V_2_dot : sym (value not decoded)
  V_3 : sym (value not decoded)
  V_3_dot : sym (value not decoded)
  V_4 : sym (value not decoded)
  V_4_dot : sym (value not decoded)
  V_5 : sym (value not decoded)
  V_5_dot : sym (value not decoded)
  V_6 : sym (value not decoded)
  V_6_dot : sym (value not decoded)
  V_7 : sym (value not decoded)
  V_7_dot : sym (value not decoded)
  V_C_1_dot : sym (value not decoded)
  V_C_2_dot : sym (value not decoded)
  V_C_3_dot : sym (value not decoded)
  V_C_4_dot : sym (value not decoded)
  V_C_5_dot : sym (value not decoded)
  V_C_6_dot : sym (value not decoded)
  V_C_7_dot : sym (value not decoded)
  Var1 = 0
  W_0 = [0; 0; 0]
  W_0_dot = [0; 0; 0]
  W_1 : sym (value not decoded)
  W_1_dot : sym (value not decoded)
  W_2 : sym (value not decoded)
  W_2_dot : sym (value not decoded)
  W_3 : sym (value not decoded)
  W_3_dot : sym (value not decoded)
  W_4 : sym (value not decoded)
  W_4_dot : sym (value not decoded)
  W_5 : sym (value not decoded)
  W_5_dot : sym (value not decoded)
  W_6 : sym (value not decoded)
  W_6_dot : sym (value not decoded)
  W_7 : sym (value not decoded)
  W_7_dot : sym (value not decoded)
  a_0 = 0
  a_1 = 0
  a_2 = 0
  a_3 = 0
  a_4 = 0
  a_5 = 0
  a_6 = 0
  a_7 = 0
  alpha_0 = 0
  alpha_1 = 90
  alpha_2 = -90
  alpha_3 = -90
  alpha_4 = 90
  alpha_5 = 90
  alpha_6 = -90
  alpha_7 = 0
  d_1 = 0
  d_2 = 0
  d_3 = 0.4
  d_4 = 0
  d_5 = 0.39
  d_6 = 0
  d_7 = 0
  d_8 = 0
  f1 = sym
  f1.s : char (value not decoded)
  f2 = sym
  f2.s : char (value not decoded)
  f3 = sym
  f3.s : char (value not decoded)
  f4 = sym
  f4.s : char (value not decoded)
  f5 = sym
  f5.s : char (value not decoded)
  f6 = sym
  f6.s : char (value not decoded)
  f7 : sym (value not decoded)
  f_end = [0; 0; 0]
  g : sym (value not decoded)
  m1 = 3.94781
  m2 = 4.50275
  m3 = 2.4552
  m4 = 2.61155
  m5 = 3.41
  m6 = 3.38795
  m7 = 0.35432
  n1 = sym
  n1.s : char (value not decoded)
  n2 = sym
  n2.s : char (value not decoded)
  n3 = sym
  n3.s : char (value not decoded)
  n4 : sym (value not decoded)
  n5 : sym (value not decoded)
  n6 : sym (value not decoded)
  n7 : sym (value not decoded)
  n_end = [0; 0; 0]
  pi = 180
  q_1 : sym (value not decoded)
  q_1_ddot : sym (value not decoded)
  q_1_dot : sym (value not decoded)
  q_2 : sym (value not decoded)
  q_2_ddot : sym (value not decoded)
  q_2_dot : sym (value not decoded)
  q_3 : sym (value not decoded)
  q_3_ddot : sym (value not decoded)
  q_3_dot : sym (value not decoded)
  q_4 : sym (value not decoded)
  q_4_ddot : sym (value not decoded)
  q_4_dot : sym (value not decoded)
  q_5 : sym (value not decoded)
  q_5_ddot : sym (value not decoded)
  q_5_dot : sym (value not decoded)
  q_6 : sym (value not decoded)
  q_6_ddot : sym (value not decoded)
  q_6_dot : sym (value not decoded)
  q_7 : sym (value not decoded)
  q_7_ddot : sym (value not decoded)
  q_7_dot : sym (value not decoded)
  thau_1 : sym (value not decoded)
  thau_2 : sym (value not decoded)
  thau_3 : sym (value not decoded)
  thau_4 : sym (value not decoded)
  thau_5 : sym (value not decoded)
  thau_6 : sym (value not decoded)
  thau_7 : sym (value not decoded)
  theta_1 : sym (value not decoded)
  theta_2 : sym (value not decoded)
  theta_3 : sym (value not decoded)
  theta_4 : sym (value not decoded)
  theta_5 : sym (value not decoded)
  theta_6 : sym (value not decoded)
  theta_7 : sym (value not decoded)
  theta_8 = 0
(part 1 of 2)
settings Model: Creator=AMIN  LastModifiedBy=SEPEHR
settings DebuggingCC: LibraryContextMissingDiagnostic=none
settings SFSimCC: SimUseLocalCustomCode=off
settings RTWCC: RTWUseLocalCustomCode=off

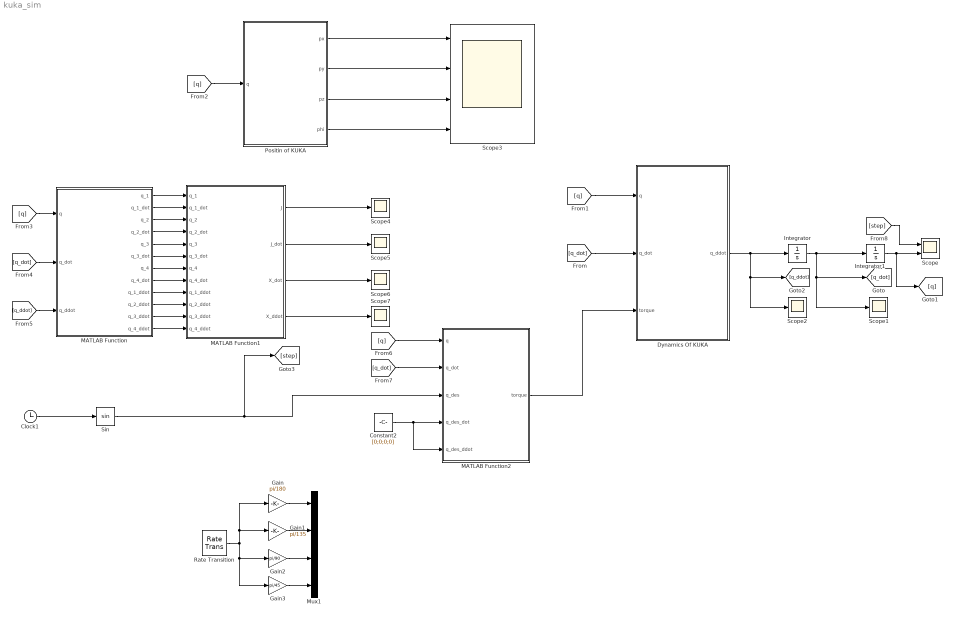
== system kuka_sim ==
  Clock1 : Clock
  Constant2 : Constant  Value=[0;0;0;0]
  Dynamics Of KUKA : MATLAB Function  TreatAsAtomicUnit=on
  Gain : Gain  Gain=pi/180
  Gain1 : Gain  Gain=pi/135
  Gain2 : Gain  Gain=pi/90
  Gain3 : Gain  Gain=pi/45
  Integrator : Integrator  InitialCondition=[0;0;0;0;]
  Integrator1 : Integrator  InitialCondition=[1;1;1;1]
  MATLAB Function : MATLAB Function  TreatAsAtomicUnit=on
  MATLAB Function1 : MATLAB Function  TreatAsAtomicUnit=on
  MATLAB Function2 : MATLAB Function  TreatAsAtomicUnit=on
  Mux1 : Mux
  "Positin of KUKA " : MATLAB Function  TreatAsAtomicUnit=on
  Rate Transition : RateTransition  OutPortSampleTime=4
  Scope : Scope  NumInputPorts=2
  Scope{1..2,4..7} (6 alike) : Scope
  Scope3 : Scope  NumInputPorts=4
  Sin : Trigonometry
  wires:
  Integrator1/1 -> [q], Scope/2
  [q_dot] -> Dynamics Of KUKA/2(q_dot)
  Dynamics Of KUKA/1(q_ddot) -> Integrator/1, [q_ddot], Scope2/1
  Integrator/1 -> Integrator1/1, Scope1/1, [q_dot]
  [q] -> Dynamics Of KUKA/1(q)
  [q] -> "Positin of KUKA "/1(q)
  "Positin of KUKA "/4(phi) -> Scope3/4
  "Positin of KUKA "/3(pz) -> Scope3/3
  "Positin of KUKA "/2(py) -> Scope3/2
  "Positin of KUKA "/1(px) -> Scope3/1
  MATLAB Function/1(q_1) -> MATLAB Function1/1(q_1)
  MATLAB Function/2(q_1_dot) -> MATLAB Function1/2(q_1_dot)
  MATLAB Function/3(q_2) -> MATLAB Function1/3(q_2)
  MATLAB Function/4(q_2_dot) -> MATLAB Function1/4(q_2_dot)
  MATLAB Function/5(q_3) -> MATLAB Function1/5(q_3)
  MATLAB Function/6(q_3_dot) -> MATLAB Function1/6(q_3_dot)
  MATLAB Function/7(q_4) -> MATLAB Function1/7(q_4)
  MATLAB Function/9(q_1_ddot) -> MATLAB Function1/9(q_1_ddot)
  MATLAB Function/10(q_2_ddot) -> MATLAB Function1/10(q_2_ddot)
  MATLAB Function/11(q_3_ddot) -> MATLAB Function1/11(q_3_ddot)
  MATLAB Function/8(q_4_dot) -> MATLAB Function1/8(q_4_dot)
  MATLAB Function/12(q_4_ddot) -> MATLAB Function1/12(q_4_ddot)
  [q] -> MATLAB Function/1(q)
  [q_dot] -> MATLAB Function/2(q_dot)
  [q_ddot] -> MATLAB Function/3(q_ddot)
  MATLAB Function1/4(X_ddot) -> Scope7/1
  MATLAB Function1/3(X_dot) -> Scope6/1
  MATLAB Function1/2(J_dot) -> Scope5/1
  MATLAB Function1/1(J) -> Scope4/1
  [q] -> MATLAB Function2/1(q)
  [q_dot] -> MATLAB Function2/2(q_dot)
  Constant2/1 -> MATLAB Function2/5(q_des_ddot), MATLAB Function2/4(q_des_dot)
  Gain2/1 -> Mux1/3
  Gain/1 -> Mux1/1
  Gain1/1 -> Mux1/2
  Rate Transition/1 -> Gain1/1, Gain/1, Gain2/1, Gain3/1
  Gain3/1 -> Mux1/4
  MATLAB Function2/1(torque) -> Dynamics Of KUKA/3(torque)
  [step] -> Scope/1
  Clock1/1 -> Sin/1
  Sin/1 -> [step], MATLAB Function2/3(q_des)

== matlab function kuka_sim/Positin of KUKA  ==
  data: q input; px output; py output; pz output; phi output
function [px,py,pz,phi] = fcn(q)
%#codegen

q_1 = q(1);
q_2 = q(2);
q_3 = q(3);
q_4 = q(4);

px = -0.4*cos(q_1)*sin(q_2)
py = -0.4*sin(q_1)*sin(q_2)
pz = 0.4*cos(q_2);
phi = q(1) + q(2) + q(3) + q(4);

== matlab function kuka_sim/Dynamics Of KUKA ==
  data: q input; q_dot input; torque input; q_ddot output
function q_ddot = fcn(q,q_dot,torque)

q_1=q(1);
q_2=q(2);
q_3=q(3);
q_4=q(4);

q_1_dot=q_dot(1);
q_2_dot=q_dot(2);
q_3_dot=q_dot(3);
q_4_dot=q_dot(4);


m11=cos(q_2)*(0.00415795377963*cos(q_2) + 0.005756821258825*sin(q_2) + 0.001993178216*cos(q_3)*sin(q_2) - 0.03195052591232*sin(q_2)*sin(q_3) + 1.0*cos(q_4)*(0.01524699328022*cos(q_2)*cos(q_4) - 0.000208924*cos(q_3)*sin(q_2) - 0.0008524847092*cos(q_2)*sin(q_4) + 0.00414266901372*sin(q_2)*sin(q_3) + 0.0008524847092*cos(q_3)*cos(q_4)*sin(q_2) + 0.01524699328022*cos(q_3)*sin(q_2)*sin(q_4) + 0.0398835916*cos(q_4)*sin(q_2)*sin(q_3)) + sin(q_4)*(0.0009075152908*cos(q_2)*cos(q_4) - 0.0550305816*cos(q_3)*sin(q_2) + 0.04949441641494*cos(q_2)*sin(q_4) - 0.0011399417958*sin(q_2)*sin(q_3) + 0.0398835916*sin(q_2)*sin(q_3)*sin(q_4) - 0.04949441641494*cos(q_3)*cos(q_4)*sin(q_2) + 0.0009075152908*cos(q_3)*sin(q_2)*sin(q_4))) + 1.0*sin(q_2)*(0.005756821258825*cos(q_2) + 0.12548815863615*sin(q_2) - 1.0*cos(q_3)*(0.000076501784*cos(q_2) + 0.01909410731264*cos(q_3)*sin(q_2) - 0.000242905064*sin(q_2)*sin(q_3) + 1.0*cos(q_4)*(0.0009075152908*cos(q_2)*cos(q_4) - 0.0550305816*cos(q_3)*sin(q_2) + 0.04949441641494*cos(q_2)*sin(q_4) - 0.0011399417958*sin(q_2)*sin(q_3) + 0.0398835916*sin(q_2)*sin(q_3)*sin(q_4) - 0.04949441641494*cos(q_3)*cos(q_4)*sin(q_2) + 0.0009075152908*cos(q_3)*sin(q_2)*sin(q_4)) - 1.0*sin(q_4)*(0.01524699328022*cos(q_2)*cos(q_4) - 0.000208924*cos(q_3)*sin(q_2) - 0.0008524847092*cos(q_2)*sin(q_4) + 0.00414266901372*sin(q_2)*sin(q_3) + 0.0008524847092*cos(q_3)*cos(q_4)*sin(q_2) + 0.01524699328022*cos(q_3)*sin(q_2)*sin(q_4) + 0.0398835916*cos(q_4)*sin(q_2)*sin(q_3))) + 1.0*sin(q_3)*(0.00220370768768*cos(q_2) + 0.00636266901372*cos(q_2)*cos(q_4) + 0.000142905064*cos(q_3)*sin(q_2) + 0.0011000582042*cos(q_2)*sin(q_4) + 0.0350120676028*sin(q_2)*sin(q_3) - 0.000208924*sin(q_2)*sin(q_3)*sin(q_4) - 0.0011000582042*cos(q_3)*cos(q_4)*sin(q_2) + 0.00636266901372*cos(q_3)*sin(q_2)*sin(q_4) + 0.0550305816*cos(q_4)*sin(q_2)*sin(q_3)) + 0.4*sin(q_3)*(cos(q_4)*(0.099708979*cos(q_2)*cos(q_4) + 0.137576454*sin(q_2)*sin(q_3) + 0.099708979*cos(q_3)*sin(q_2)*sin(q_4) + 1.04462*cos(q_4)*sin(q_2)*sin(q_3)) - 0.085735584*cos(q_2) + 0.916968096*sin(q_2)*sin(q_3) + 1.0*sin(q_4)*(0.099708979*cos(q_2)*sin(q_4) - 0.00052231*sin(q_2)*sin(q_3) + 1.04462*sin(q_2)*sin(q_3)*sin(q_4) - 0.099708979*cos(q_3)*cos(q_4)*sin(q_2))) + 0.4*cos(q_3)*(0.0055242*cos(q_2) - 0.00052231*cos(q_2)*cos(q_4) + 1.961588096*cos(q_3)*sin(q_2) - 0.137576454*cos(q_2)*sin(q_4) + 0.137576454*cos(q_3)*cos(q_4)*sin(q_2) - 0.00052231*cos(q_3)*sin(q_2)*sin(q_4))) + 0.00034874380758100000061534551321074;
m12=1.0*sin(q_2)*(1.0*cos(q_3)*(0.000242905064*cos(q_3) + 0.01909410731264*sin(q_3) - 1.0*cos(q_4)*(0.0550305816*sin(q_3) - 0.0011399417958*cos(q_3) + 0.0398835916*cos(q_3)*sin(q_4) + 0.04949441641494*cos(q_4)*sin(q_3) - 0.0009075152908*sin(q_3)*sin(q_4)) + 1.0*sin(q_4)*(0.00414266901372*cos(q_3) + 0.000208924*sin(q_3) + 0.0398835916*cos(q_3)*cos(q_4) - 0.0008524847092*cos(q_4)*sin(q_3) - 0.01524699328022*sin(q_3)*sin(q_4))) - 0.4*cos(q_3)*(1.961588096*sin(q_3) + 0.137576454*cos(q_4)*sin(q_3) - 0.00052231*sin(q_3)*sin(q_4)) + 0.4*sin(q_3)*(0.916968096*cos(q_3) + cos(q_4)*(0.137576454*cos(q_3) + 1.04462*cos(q_3)*cos(q_4) - 0.099708979*sin(q_3)*sin(q_4)) + 1.0*sin(q_4)*(1.04462*cos(q_3)*sin(q_4) - 0.00052231*cos(q_3) + 0.099708979*cos(q_4)*sin(q_3))) + 1.0*sin(q_3)*(0.0350120676028*cos(q_3) - 0.000142905064*sin(q_3) + 0.0550305816*cos(q_3)*cos(q_4) - 0.000208924*cos(q_3)*sin(q_4) + 0.0011000582042*cos(q_4)*sin(q_3) - 0.00636266901372*sin(q_3)*sin(q_4)) - 0.000122603128375) + cos(q_2)*(1.0*cos(q_4)*(0.00414266901372*cos(q_3) + 0.000208924*sin(q_3) + 0.0398835916*cos(q_3)*cos(q_4) - 0.0008524847092*cos(q_4)*sin(q_3) - 0.01524699328022*sin(q_3)*sin(q_4)) - 0.001993178216*sin(q_3) - 0.03195052591232*cos(q_3) + sin(q_4)*(0.0550305816*sin(q_3) - 0.0011399417958*cos(q_3) + 0.0398835916*cos(q_3)*sin(q_4) + 0.04949441641494*cos(q_4)*sin(q_3) - 0.0009075152908*sin(q_3)*sin(q_4)) + 0.002664500061125);
m13=cos(q_2)*(sin(q_4)*(0.0009075152908*cos(q_4) + 0.04949441641494*sin(q_4)) + 1.0*cos(q_4)*(0.01524699328022*cos(q_4) - 0.0008524847092*sin(q_4)) + 0.00373631604328) + 1.0*sin(q_2)*(1.0*sin(q_3)*(0.00636266901372*cos(q_4) + 0.0011000582042*sin(q_4) + 0.00220370768768) - 1.0*cos(q_3)*(1.0*cos(q_4)*(0.0009075152908*cos(q_4) + 0.04949441641494*sin(q_4)) - 1.0*sin(q_4)*(0.01524699328022*cos(q_4) - 0.0008524847092*sin(q_4)) + 0.000076501784) - 0.4*cos(q_3)*(0.00052231*cos(q_4) + 0.137576454*sin(q_4) - 0.0055242) + 0.4*sin(q_3)*(0.099708979*cos(q_4)^2 + 0.099708979*sin(q_4)^2 - 0.085735584));
m14=- 1.0*sin(q_2)*(0.05712763205872*sin(q_3) + 1.0*cos(q_3)*(0.0011399417958*cos(q_4) + 0.00414266901372*sin(q_4)) + 0.4*sin(q_3)*(0.137576454*cos(q_4) - 0.00052231*sin(q_4))) - cos(q_2)*(0.00414266901372*cos(q_4) - 0.0011399417958*sin(q_4));
m21=0.002664500061125*cos(q_2) - 0.000122603128375*sin(q_2) + sin(q_3)*(0.000076501784*cos(q_2) + 0.01909410731264*cos(q_3)*sin(q_2) - 0.000242905064*sin(q_2)*sin(q_3) + 1.0*cos(q_4)*(0.0009075152908*cos(q_2)*cos(q_4) - 0.0550305816*cos(q_3)*sin(q_2) + 0.04949441641494*cos(q_2)*sin(q_4) - 0.0011399417958*sin(q_2)*sin(q_3) + 0.0398835916*sin(q_2)*sin(q_3)*sin(q_4) - 0.04949441641494*cos(q_3)*cos(q_4)*sin(q_2) + 0.0009075152908*cos(q_3)*sin(q_2)*sin(q_4)) - 1.0*sin(q_4)*(0.01524699328022*cos(q_2)*cos(q_4) - 0.000208924*cos(q_3)*sin(q_2) - 0.0008524847092*cos(q_2)*sin(q_4) + 0.00414266901372*sin(q_2)*sin(q_3) + 0.0008524847092*cos(q_3)*cos(q_4)*sin(q_2) + 0.01524699328022*cos(q_3)*sin(q_2)*sin(q_4) + 0.0398835916*cos(q_4)*sin(q_2)*sin(q_3))) + 1.0*cos(q_3)*(0.00220370768768*cos(q_2) + 0.00636266901372*cos(q_2)*cos(q_4) + 0.000142905064*cos(q_3)*sin(q_2) + 0.0011000582042*cos(q_2)*sin(q_4) + 0.0350120676028*sin(q_2)*sin(q_3) - 0.000208924*sin(q_2)*sin(q_3)*sin(q_4) - 0.0011000582042*cos(q_3)*cos(q_4)*sin(q_2) + 0.00636266901372*cos(q_3)*sin(q_2)*sin(q_4) + 0.0550305816*cos(q_4)*sin(q_2)*sin(q_3)) + 0.4*cos(q_3)*(cos(q_4)*(0.099708979*cos(q_2)*cos(q_4) + 0.137576454*sin(q_2)*sin(q_3) + 0.099708979*cos(q_3)*sin(q_2)*sin(q_4) + 1.04462*cos(q_4)*sin(q_2)*sin(q_3)) - 0.085735584*cos(q_2) + 0.916968096*sin(q_2)*sin(q_3) + 1.0*sin(q_4)*(0.099708979*cos(q_2)*sin(q_4) - 0.00052231*sin(q_2)*sin(q_3) + 1.04462*sin(q_2)*sin(q_3)*sin(q_4) - 0.099708979*cos(q_3)*cos(q_4)*sin(q_2))) - 0.4*sin(q_3)*(0.0055242*cos(q_2) - 0.00052231*cos(q_2)*cos(q_4) + 1.961588096*cos(q_3)*sin(q_2) - 0.137576454*cos(q_2)*sin(q_4) + 0.137576454*cos(q_3)*cos(q_4)*sin(q_2) - 0.00052231*cos(q_3)*sin(q_2)*sin(q_4));
m22=0.4*sin(q_3)*(1.961588096*sin(q_3) + 0.137576454*cos(q_4)*sin(q_3) - 0.00052231*sin(q_3)*sin(q_4)) - sin(q_3)*(0.000242905064*cos(q_3) + 0.01909410731264*sin(q_3) - 1.0*cos(q_4)*(0.0550305816*sin(q_3) - 0.0011399417958*cos(q_3) + 0.0398835916*cos(q_3)*sin(q_4) + 0.04949441641494*cos(q_4)*sin(q_3) - 0.0009075152908*sin(q_3)*sin(q_4)) + 1.0*sin(q_4)*(0.00414266901372*cos(q_3) + 0.000208924*sin(q_3) + 0.0398835916*cos(q_3)*cos(q_4) - 0.0008524847092*cos(q_4)*sin(q_3) - 0.01524699328022*sin(q_3)*sin(q_4))) + 0.4*cos(q_3)*(0.916968096*cos(q_3) + cos(q_4)*(0.137576454*cos(q_3) + 1.04462*cos(q_3)*cos(q_4) - 0.099708979*sin(q_3)*sin(q_4)) + 1.0*sin(q_4)*(1.04462*cos(q_3)*sin(q_4) - 0.00052231*cos(q_3) + 0.099708979*cos(q_4)*sin(q_3))) + 1.0*cos(q_3)*(0.0350120676028*cos(q_3) - 0.000142905064*sin(q_3) + 0.0550305816*cos(q_3)*cos(q_4) - 0.000208924*cos(q_3)*sin(q_4) + 0.0011000582042*cos(q_4)*sin(q_3) - 0.00636266901372*sin(q_3)*sin(q_4)) + 0.12579630455875;
m23=0.4*sin(q_3)*(0.00052231*cos(q_4) + 0.137576454*sin(q_4) - 0.0055242) + 1.0*cos(q_3)*(0.00636266901372*cos(q_4) + 0.0011000582042*sin(q_4) + 0.00220370768768) + sin(q_3)*(1.0*cos(q_4)*(0.0009075152908*cos(q_4) + 0.04949441641494*sin(q_4)) - 1.0*sin(q_4)*(0.01524699328022*cos(q_4) - 0.0008524847092*sin(q_4)) + 0.000076501784) + 0.4*cos(q_3)*(0.099708979*cos(q_4)^2 + 0.099708979*sin(q_4)^2 - 0.085735584);
m24=sin(q_3)*(0.0011399417958*cos(q_4) + 0.00414266901372*sin(q_4)) - 0.4*cos(q_3)*(0.137576454*cos(q_4) - 0.00052231*sin(q_4)) - 0.05712763205872*cos(q_3);
m31=0.00373631604328*cos(q_2) + 0.001993178216*cos(q_3)*sin(q_2) - 0.03195052591232*sin(q_2)*sin(q_3) + 1.0*cos(q_4)*(0.01524699328022*cos(q_2)*cos(q_4) - 0.000208924*cos(q_3)*sin(q_2) - 0.0008524847092*cos(q_2)*sin(q_4) + 0.00414266901372*sin(q_2)*sin(q_3) + 0.0008524847092*cos(q_3)*cos(q_4)*sin(q_2) + 0.01524699328022*cos(q_3)*sin(q_2)*sin(q_4) + 0.0398835916*cos(q_4)*sin(q_2)*sin(q_3)) + sin(q_4)*(0.0009075152908*cos(q_2)*cos(q_4) - 0.0550305816*cos(q_3)*sin(q_2) + 0.04949441641494*cos(q_2)*sin(q_4) - 0.0011399417958*sin(q_2)*sin(q_3) + 0.0398835916*sin(q_2)*sin(q_3)*sin(q_4) - 0.04949441641494*cos(q_3)*cos(q_4)*sin(q_2) + 0.0009075152908*cos(q_3)*sin(q_2)*sin(q_4));
m32=1.0*cos(q_4)*(0.00414266901372*cos(q_3) + 0.000208924*sin(q_3) + 0.0398835916*cos(q_3)*cos(q_4) - 0.0008524847092*cos(q_4)*sin(q_3) - 0.01524699328022*sin(q_3)*sin(q_4)) - 0.001993178216*sin(q_3) - 0.03195052591232*cos(q_3) + sin(q_4)*(0.0550305816*sin(q_3) - 0.0011399417958*cos(q_3) + 0.0398835916*cos(q_3)*sin(q_4) + 0.04949441641494*cos(q_4)*sin(q_3) - 0.0009075152908*sin(q_3)*sin(q_4));
m33=sin(q_4)*(0.0009075152908*cos(q_4) + 0.04949441641494*sin(q_4)) + 1.0*cos(q_4)*(0.01524699328022*cos(q_4) - 0.0008524847092*sin(q_4)) + 0.00373631604328;
m34=0.0011399417958*sin(q_4) - 0.00414266901372*cos(q_4);
m41=0.000208924*sin(q_2)*sin(q_3)*sin(q_4) - 0.0011000582042*cos(q_2)*sin(q_4) - 0.05712763205872*sin(q_2)*sin(q_3) - 0.00636266901372*cos(q_2)*cos(q_4) + 0.0011000582042*cos(q_3)*cos(q_4)*sin(q_2) - 0.00636266901372*cos(q_3)*sin(q_2)*sin(q_4) - 0.0550305816*cos(q_4)*sin(q_2)*sin(q_3);
m42=0.000208924*cos(q_3)*sin(q_4) - 0.0550305816*cos(q_3)*cos(q_4) - 0.05712763205872*cos(q_3) - 0.0011000582042*cos(q_4)*sin(q_3) + 0.00636266901372*sin(q_3)*sin(q_4);
m43=- 0.00636266901372*cos(q_4) - 0.0011000582042*sin(q_4);
m44=0.05712763205872;

% M=[m11 m12 m13 m14;m21 m22 m23 m24;m31 m32 m33 m34;m41 m42 m43 m44 ];

%c
c11=0;
c12=- cos(q_2)*(0.005756821258825*q_1*sin(q_2)^2 + 0.0055242*cos(q_3)*(0.4*q_1*sin(q_2)^2 - 0.4*q_2*cos(q_2)) - 0.085735584*sin(q_3)*(0.4*q_1*sin(q_2)^2 - 0.4*q_2*cos(q_2)) + 1.0*cos(q_4)*(0.01524699328022*cos(q_4)*(1.0*q_2*sin(q_2) + 1.0*q_1*cos(q_2)*sin(q_2)) - 0.00052231*cos(q_3)*(0.4*q_1*sin(q_2)^2 - 0.4*q_2*cos(q_2)) - 0.0008524847092*sin(q_4)*(1.0*q_2*sin(q_2) + 1.0*q_1*cos(q_2)*sin(q_2)) + 0.00414266901372*sin(q_3)*(1.0*q_1*sin(q_2)^2 - 1.0*q_2*cos(q_2)) + 0.0008524847092*cos(q_3)*cos(q_4)*(1.0*q_1*sin(q_2)^2 - 1.0*q_2*cos(q_2)) + 0.01524699328022*cos(q_3)*sin(q_4)*(1.0*q_1*sin(q_2)^2 - 1.0*q_2*cos(q_2)) + 0.099708979*cos(q_4)*sin(q_3)*(0.4*q_1*sin(q_2)^2 - 0.4*q_2*cos(q_2))) + sin(q_4)*(0.0009075152908*cos(q_4)*(1.0*q_2*sin(q_2) + 1.0*q_1*cos(q_2)*sin(q_2)) - 0.137576454*cos(q_3)*(0.4*q_1*sin(q_2)^2 - 0.4*q_2*cos(q_2)) + 0.04949441641494*sin(q_4)*(1.0*q_2*sin(q_2) + 1.0*q_1*cos(q_2)*sin(q_2)) - 0.0011399417958*sin(q_3)*(1.0*q_1*sin(q_2)^2 - 1.0*q_2*cos(q_2)) + 0.099708979*sin(q_3)*sin(q_4)*(0.4*q_1*sin(q_2)^2 - 0.4*q_2*cos(q_2)) - 0.04949441641494*cos(q_3)*cos(q_4)*(1.0*q_1*sin(q_2)^2 - 1.0*q_2*cos(q_2)) + 0.0009075152908*cos(q_3)*sin(q_4)*(1.0*q_1*sin(q_2)^2 - 1.0*q_2*cos(q_2))) - 0.005756821258825*q_2*cos(q_2) + 0.00415795377963*q_2*sin(q_2) - 0.000216501784*cos(q_3)*(1.0*q_1*sin(q_2)^2 - 1.0*q_2*cos(q_2)) + 0.00234370768768*sin(q_3)*(1.0*q_1*sin(q_2)^2 - 1.0*q_2*cos(q_2)) + 0.00415795377963*q_1*cos(q_2)*sin(q_2)) - 1.0*sin(q_2)*(0.12548815863615*q_1*sin(q_2)^2 + 0.4*cos(q_3)*(5.06675*cos(q_3)*(0.4*q_1*sin(q_2)^2 - 0.4*q_2*cos(q_2)) - 0.00052231*cos(q_4)*(1.0*q_2*sin(q_2) + 1.0*q_1*cos(q_2)*sin(q_2)) - 0.137576454*sin(q_4)*(1.0*q_2*sin(q_2) + 1.0*q_1*cos(q_2)*sin(q_2)) + 0.0055242*q_2*sin(q_2) - 0.065111904*cos(q_3)*(1.0*q_1*sin(q_2)^2 - 1.0*q_2*cos(q_2)) + 0.0055242*q_1*cos(q_2)*sin(q_2) + 0.137576454*cos(q_3)*cos(q_4)*(1.0*q_1*sin(q_2)^2 - 1.0*q_2*cos(q_2)) - 0.00052231*cos(q_3)*sin(q_4)*(1.0*q_1*sin(q_2)^2 - 1.0*q_2*cos(q_2))) + 0.4*sin(q_3)*(2.4552*sin(q_3)*(0.4*q_1*sin(q_2)^2 - 0.4*q_2*cos(q_2)) - 0.085735584*q_2*sin(q_2) - 0.065111904*sin(q_3)*(1.0*q_1*sin(q_2)^2 - 1.0*q_2*cos(q_2)) + cos(q_4)*(0.099708979*cos(q_4)*(1.0*q_2*sin(q_2) + 1.0*q_1*cos(q_2)*sin(q_2)) + 0.137576454*sin(q_3)*(1.0*q_1*sin(q_2)^2 - 1.0*q_2*cos(q_2)) + 0.099708979*cos(q_3)*sin(q_4)*(1.0*q_1*sin(q_2)^2 - 1.0*q_2*cos(q_2)) + 2.61155*cos(q_4)*sin(q_3)*(0.4*q_1*sin(q_2)^2 - 0.4*q_2*cos(q_2))) + 1.0*sin(q_4)*(0.099708979*sin(q_4)*(1.0*q_2*sin(q_2) + 1.0*q_1*cos(q_2)*sin(q_2)) - 0.00052231*sin(q_3)*(1.0*q_1*sin(q_2)^2 - 1.0*q_2*cos(q_2)) + 2.61155*sin(q_3)*sin(q_4)*(0.4*q_1*sin(q_2)^2 - 0.4*q_2*cos(q_2)) - 0.099708979*cos(q_3)*cos(q_4)*(1.0*q_1*sin(q_2)^2 - 1.0*q_2*cos(q_2))) - 0.085735584*q_1*cos(q_2)*sin(q_2)) + 1.0*sin(q_3)*(0.00636266901372*cos(q_4)*(1.0*q_2*sin(q_2) + 1.0*q_1*cos(q_2)*sin(q_2)) - 0.065111904*sin(q_3)*(0.4*q_1*sin(q_2)^2 - 0.4*q_2*cos(q_2)) + 0.0011000582042*sin(q_4)*(1.0*q_2*sin(q_2) + 1.0*q_1*cos(q_2)*sin(q_2)) + 0.00220370768768*q_2*sin(q_2) + 0.000142905064*cos(q_3)*(1.0*q_1*sin(q_2)^2 - 1.0*q_2*cos(q_2)) + 0.0610568292028*sin(q_3)*(1.0*q_1*sin(q_2)^2 - 1.0*q_2*cos(q_2)) - 0.00052231*sin(q_3)*sin(q_4)*(0.4*q_1*sin(q_2)^2 - 0.4*q_2*cos(q_2)) + 0.00220370768768*q_1*cos(q_2)*sin(q_2) - 0.0011000582042*cos(q_3)*cos(q_4)*(1.0*q_1*sin(q_2)^2 - 1.0*q_2*cos(q_2)) + 0.00636266901372*cos(q_3)*sin(q_4)*(1.0*q_1*sin(q_2)^2 - 1.0*q_2*cos(q_2)) + 0.137576454*cos(q_4)*sin(q_3)*(0.4*q_1*sin(q_2)^2 - 0.4*q_2*cos(q_2))) - 0.12548815863615*q_2*cos(q_2) + 0.005756821258825*q_2*sin(q_2) - 1.0*cos(q_3)*(0.065111904*cos(q_3)*(0.4*q_1*sin(q_2)^2 - 0.4*q_2*cos(q_2)) + 1.0*cos(q_4)*(0.0009075152908*cos(q_4)*(1.0*q_2*sin(q_2) + 1.0*q_1*cos(q_2)*sin(q_2)) - 0.137576454*cos(q_3)*(0.4*q_1*sin(q_2)^2 - 0.4*q_2*cos(q_2)) + 0.04949441641494*sin(q_4)*(1.0*q_2*sin(q_2) + 1.0*q_1*cos(q_2)*sin(q_2)) - 0.0011399417958*sin(q_3)*(1.0*q_1*sin(q_2)^2 - 1.0*q_2*cos(q_2)) + 0.099708979*sin(q_3)*sin(q_4)*(0.4*q_1*sin(q_2)^2 - 0.4*q_2*cos(q_2)) - 0.04949441641494*cos(q_3)*cos(q_4)*(1.0*q_1*sin(q_2)^2 - 1.0*q_2*cos(q_2)) + 0.0009075152908*cos(q_3)*sin(q_4)*(1.0*q_1*sin(q_2)^2 - 1.0*q_2*cos(q_2))) - 1.0*sin(q_4)*(0.01524699328022*cos(q_4)*(1.0*q_2*sin(q_2) + 1.0*q_1*cos(q_2)*sin(q_2)) - 0.00052231*cos(q_3)*(0.4*q_1*sin(q_2)^2 - 0.4*q_2*cos(q_2)) - 0.0008524847092*sin(q_4)*(1.0*q_2*sin(q_2) + 1.0*q_1*cos(q_2)*sin(q_2)) + 0.00414266901372*sin(q_3)*(1.0*q_1*sin(q_2)^2 - 1.0*q_2*cos(q_2)) + 0.0008524847092*cos(q_3)*cos(q_4)*(1.0*q_1*sin(q_2)^2 - 1.0*q_2*cos(q_2)) + 0.01524699328022*cos(q_3)*sin(q_4)*(1.0*q_1*sin(q_2)^2 - 1.0*q_2*cos(q_2)) + 0.099708979*cos(q_4)*sin(q_3)*(0.4*q_1*sin(q_2)^2 - 0.4*q_2*cos(q_2))) + 0.000076501784*q_2*sin(q_2) - 0.00695065428736*cos(q_3)*(1.0*q_1*sin(q_2)^2 - 1.0*q_2*cos(q_2)) - 0.000242905064*sin(q_3)*(1.0*q_1*sin(q_2)^2 - 1.0*q_2*cos(q_2)) + 0.000076501784*q_1*cos(q_2)*sin(q_2)) + 0.005756821258825*q_1*cos(q_2)*sin(q_2));
c13=- 1.0*sin(q_2)*(0.4*cos(q_3)*(0.065111904*sin(q_3)*(q_2*sin(q_3) - 1.0*q_1*cos(q_3)*sin(q_2)) - 0.065111904*cos(q_3)*(q_3 + q_1*cos(q_2)) - 0.137576454*cos(q_4)*(1.0*sin(q_3)*(q_2*sin(q_3) - 1.0*q_1*cos(q_3)*sin(q_2)) - 1.0*cos(q_3)*(q_3 + q_1*cos(q_2))) + 0.00052231*sin(q_4)*(1.0*sin(q_3)*(q_2*sin(q_3) - 1.0*q_1*cos(q_3)*sin(q_2)) - 1.0*cos(q_3)*(q_3 + q_1*cos(q_2)))) + 1.0*sin(q_3)*(0.0610568292028*cos(q_3)*(q_2*sin(q_3) - 1.0*q_1*cos(q_3)*sin(q_2)) - 0.000142905064*sin(q_3)*(q_2*sin(q_3) - 1.0*q_1*cos(q_3)*sin(q_2)) + 0.000142905064*cos(q_3)*(q_3 + q_1*cos(q_2)) + 0.0610568292028*sin(q_3)*(q_3 + q_1*cos(q_2)) + 0.0011000582042*cos(q_4)*(1.0*sin(q_3)*(q_2*sin(q_3) - 1.0*q_1*cos(q_3)*sin(q_2)) - 1.0*cos(q_3)*(q_3 + q_1*cos(q_2))) - 0.00636266901372*sin(q_4)*(1.0*sin(q_3)*(q_2*sin(q_3) - 1.0*q_1*cos(q_3)*sin(q_2)) - 1.0*cos(q_3)*(q_3 + q_1*cos(q_2)))) - 0.4*sin(q_3)*(0.065111904*cos(q_3)*(q_2*sin(q_3) - 1.0*q_1*cos(q_3)*sin(q_2)) + 1.0*sin(q_4)*(0.00052231*cos(q_3)*(q_2*sin(q_3) - 1.0*q_1*cos(q_3)*sin(q_2)) + 0.00052231*sin(q_3)*(q_3 + q_1*cos(q_2)) - 0.099708979*cos(q_4)*(1.0*sin(q_3)*(q_2*sin(q_3) - 1.0*q_1*cos(q_3)*sin(q_2)) - 1.0*cos(q_3)*(q_3 + q_1*cos(q_2)))) - cos(q_4)*(0.137576454*cos(q_3)*(q_2*sin(q_3) - 1.0*q_1*cos(q_3)*sin(q_2)) + 0.137576454*sin(q_3)*(q_3 + q_1*cos(q_2)) - 0.099708979*sin(q_4)*(1.0*sin(q_3)*(q_2*sin(q_3) - 1.0*q_1*cos(q_3)*sin(q_2)) - 1.0*cos(q_3)*(q_3 + q_1*cos(q_2)))) + 0.065111904*sin(q_3)*(q_3 + q_1*cos(q_2))) + 1.0*cos(q_3)*(0.000242905064*cos(q_3)*(q_2*sin(q_3) - 1.0*q_1*cos(q_3)*sin(q_2)) - 0.00695065428736*sin(q_3)*(q_2*sin(q_3) - 1.0*q_1*cos(q_3)*sin(q_2)) + 1.0*cos(q_4)*(0.0011399417958*cos(q_3)*(q_2*sin(q_3) - 1.0*q_1*cos(q_3)*sin(q_2)) + 0.0011399417958*sin(q_3)*(q_3 + q_1*cos(q_2)) - 0.04949441641494*cos(q_4)*(1.0*sin(q_3)*(q_2*sin(q_3) - 1.0*q_1*cos(q_3)*sin(q_2)) - 1.0*cos(q_3)*(q_3 + q_1*cos(q_2))) + 0.0009075152908*sin(q_4)*(1.0*sin(q_3)*(q_2*sin(q_3) - 1.0*q_1*cos(q_3)*sin(q_2)) - 1.0*cos(q_3)*(q_3 + q_1*cos(q_2)))) + 0.00695065428736*cos(q_3)*(q_3 + q_1*cos(q_2)) + 1.0*sin(q_4)*(0.00414266901372*cos(q_3)*(q_2*sin(q_3) - 1.0*q_1*cos(q_3)*sin(q_2)) + 0.00414266901372*sin(q_3)*(q_3 + q_1*cos(q_2)) - 0.0008524847092*cos(q_4)*(1.0*sin(q_3)*(q_2*sin(q_3) - 1.0*q_1*cos(q_3)*sin(q_2)) - 1.0*cos(q_3)*(q_3 + q_1*cos(q_2))) - 0.01524699328022*sin(q_4)*(1.0*sin(q_3)*(q_2*sin(q_3) - 1.0*q_1*cos(q_3)*sin(q_2)) - 1.0*cos(q_3)*(q_3 + q_1*cos(q_2)))) + 0.000242905064*sin(q_3)*(q_3 + q_1*cos(q_2)))) - cos(q_2)*(0.00234370768768*cos(q_3)*(q_2*sin(q_3) - 1.0*q_1*cos(q_3)*sin(q_2)) + 0.000216501784*sin(q_3)*(q_2*sin(q_3) - 1.0*q_1*cos(q_3)*sin(q_2)) + 1.0*cos(q_4)*(0.00414266901372*cos(q_3)*(q_2*sin(q_3) - 1.0*q_1*cos(q_3)*sin(q_2)) + 0.00414266901372*sin(q_3)*(q_3 + q_1*cos(q_2)) - 0.0008524847092*cos(q_4)*(1.0*sin(q_3)*(q_2*sin(q_3) - 1.0*q_1*cos(q_3)*sin(q_2)) - 1.0*cos(q_3)*(q_3 + q_1*cos(q_2))) - 0.01524699328022*sin(q_4)*(1.0*sin(q_3)*(q_2*sin(q_3) - 1.0*q_1*cos(q_3)*sin(q_2)) - 1.0*cos(q_3)*(q_3 + q_1*cos(q_2)))) - 0.000216501784*cos(q_3)*(q_3 + q_1*cos(q_2)) - sin(q_4)*(0.0011399417958*cos(q_3)*(q_2*sin(q_3) - 1.0*q_1*cos(q_3)*sin(q_2)) + 0.0011399417958*sin(q_3)*(q_3 + q_1*cos(q_2)) - 0.04949441641494*cos(q_4)*(1.0*sin(q_3)*(q_2*sin(q_3) - 1.0*q_1*cos(q_3)*sin(q_2)) - 1.0*cos(q_3)*(q_3 + q_1*cos(q_2))) + 0.0009075152908*sin(q_4)*(1.0*sin(q_3)*(q_2*sin(q_3) - 1.0*q_1*cos(q_3)*sin(q_2)) - 1.0*cos(q_3)*(q_3 + q_1*cos(q_2)))) + 0.00234370768768*sin(q_3)*(q_3 + q_1*cos(q_2)));
c14=1.0*sin(q_2)*(1.0*cos(q_3)*(1.0*sin(q_4)*(0.0008524847092*sin(q_4)*(cos(q_4)*(q_2*sin(q_3) - 1.0*q_1*cos(q_3)*sin(q_2)) + sin(q_4)*(q_3 + q_1*cos(q_2))) - 0.01524699328022*cos(q_4)*(cos(q_4)*(q_2*sin(q_3) - 1.0*q_1*cos(q_3)*sin(q_2)) + sin(q_4)*(q_3 + q_1*cos(q_2))) + 0.0008524847092*cos(q_4)*(q_2*cos(q_3) - 1.0*q_4 + q_1*sin(q_2)*sin(q_3)) + 0.01524699328022*sin(q_4)*(q_2*cos(q_3) - 1.0*q_4 + q_1*sin(q_2)*sin(q_3))) + 1.0*cos(q_4)*(0.0009075152908*cos(q_4)*(cos(q_4)*(q_2*sin(q_3) - 1.0*q_1*cos(q_3)*sin(q_2)) + sin(q_4)*(q_3 + q_1*cos(q_2))) + 0.04949441641494*sin(q_4)*(cos(q_4)*(q_2*sin(q_3) - 1.0*q_1*cos(q_3)*sin(q_2)) + sin(q_4)*(q_3 + q_1*cos(q_2))) + 0.04949441641494*cos(q_4)*(q_2*cos(q_3) - 1.0*q_4 + q_1*sin(q_2)*sin(q_3)) - 0.0009075152908*sin(q_4)*(q_2*cos(q_3) - 1.0*q_4 + q_1*sin(q_2)*sin(q_3)))) + 0.4*cos(q_3)*(0.00052231*cos(q_4)*(cos(q_4)*(q_2*sin(q_3) - 1.0*q_1*cos(q_3)*sin(q_2)) + sin(q_4)*(q_3 + q_1*cos(q_2))) + 0.137576454*sin(q_4)*(cos(q_4)*(q_2*sin(q_3) - 1.0*q_1*cos(q_3)*sin(q_2)) + sin(q_4)*(q_3 + q_1*cos(q_2))) + 0.137576454*cos(q_4)*(q_2*cos(q_3) - 1.0*q_4 + q_1*sin(q_2)*sin(q_3)) - 0.00052231*sin(q_4)*(q_2*cos(q_3) - 1.0*q_4 + q_1*sin(q_2)*sin(q_3))) - 0.4*sin(q_3)*(cos(q_4)*(0.099708979*cos(q_4)*(cos(q_4)*(q_2*sin(q_3) - 1.0*q_1*cos(q_3)*sin(q_2)) + sin(q_4)*(q_3 + q_1*cos(q_2))) - 0.099708979*sin(q_4)*(q_2*cos(q_3) - 1.0*q_4 + q_1*sin(q_2)*sin(q_3))) + 1.0*sin(q_4)*(0.099708979*sin(q_4)*(cos(q_4)*(q_2*sin(q_3) - 1.0*q_1*cos(q_3)*sin(q_2)) + sin(q_4)*(q_3 + q_1*cos(q_2))) + 0.099708979*cos(q_4)*(q_2*cos(q_3) - 1.0*q_4 + q_1*sin(q_2)*sin(q_3)))) - 1.0*sin(q_3)*(0.00636266901372*cos(q_4)*(cos(q_4)*(q_2*sin(q_3) - 1.0*q_1*cos(q_3)*sin(q_2)) + sin(q_4)*(q_3 + q_1*cos(q_2))) + 0.0011000582042*sin(q_4)*(cos(q_4)*(q_2*sin(q_3) - 1.0*q_1*cos(q_3)*sin(q_2)) + sin(q_4)*(q_3 + q_1*cos(q_2))) + 0.0011000582042*cos(q_4)*(q_2*cos(q_3) - 1.0*q_4 + q_1*sin(q_2)*sin(q_3)) - 0.00636266901372*sin(q_4)*(q_2*cos(q_3) - 1.0*q_4 + q_1*sin(q_2)*sin(q_3)))) - cos(q_2)*(sin(q_4)*(0.0009075152908*cos(q_4)*(cos(q_4)*(q_2*sin(q_3) - 1.0*q_1*cos(q_3)*sin(q_2)) + sin(q_4)*(q_3 + q_1*cos(q_2))) + 0.04949441641494*sin(q_4)*(cos(q_4)*(q_2*sin(q_3) - 1.0*q_1*cos(q_3)*sin(q_2)) + sin(q_4)*(q_3 + q_1*cos(q_2))) + 0.04949441641494*cos(q_4)*(q_2*cos(q_3) - 1.0*q_4 + q_1*sin(q_2)*sin(q_3)) - 0.0009075152908*sin(q_4)*(q_2*cos(q_3) - 1.0*q_4 + q_1*sin(q_2)*sin(q_3))) - 1.0*cos(q_4)*(0.0008524847092*sin(q_4)*(cos(q_4)*(q_2*sin(q_3) - 1.0*q_1*cos(q_3)*sin(q_2)) + sin(q_4)*(q_3 + q_1*cos(q_2))) - 0.01524699328022*cos(q_4)*(cos(q_4)*(q_2*sin(q_3) - 1.0*q_1*cos(q_3)*sin(q_2)) + sin(q_4)*(q_3 + q_1*cos(q_2))) + 0.0008524847092*cos(q_4)*(q_2*cos(q_3) - 1.0*q_4 + q_1*sin(q_2)*sin(q_3)) + 0.01524699328022*sin(q_4)*(q_2*cos(q_3) - 1.0*q_4 + q_1*sin(q_2)*sin(q_3))));
c21=0;
c22=0.000122603128375*q_1*sin(q_2)^2 + 0.4*sin(q_3)*(5.06675*cos(q_3)*(0.4*q_1*sin(q_2)^2 - 0.4*q_2*cos(q_2)) - 0.00052231*cos(q_4)*(1.0*q_2*sin(q_2) + 1.0*q_1*cos(q_2)*sin(q_2)) - 0.137576454*sin(q_4)*(1.0*q_2*sin(q_2) + 1.0*q_1*cos(q_2)*sin(q_2)) + 0.0055242*q_2*sin(q_2) - 0.065111904*cos(q_3)*(1.0*q_1*sin(q_2)^2 - 1.0*q_2*cos(q_2)) + 0.0055242*q_1*cos(q_2)*sin(q_2) + 0.137576454*cos(q_3)*cos(q_4)*(1.0*q_1*sin(q_2)^2 - 1.0*q_2*cos(q_2)) - 0.00052231*cos(q_3)*sin(q_4)*(1.0*q_1*sin(q_2)^2 - 1.0*q_2*cos(q_2))) - 0.4*cos(q_3)*(2.4552*sin(q_3)*(0.4*q_1*sin(q_2)^2 - 0.4*q_2*cos(q_2)) - 0.085735584*q_2*sin(q_2) - 0.065111904*sin(q_3)*(1.0*q_1*sin(q_2)^2 - 1.0*q_2*cos(q_2)) + cos(q_4)*(0.099708979*cos(q_4)*(1.0*q_2*sin(q_2) + 1.0*q_1*cos(q_2)*sin(q_2)) + 0.137576454*sin(q_3)*(1.0*q_1*sin(q_2)^2 - 1.0*q_2*cos(q_2)) + 0.099708979*cos(q_3)*sin(q_4)*(1.0*q_1*sin(q_2)^2 - 1.0*q_2*cos(q_2)) + 2.61155*cos(q_4)*sin(q_3)*(0.4*q_1*sin(q_2)^2 - 0.4*q_2*cos(q_2))) + 1.0*sin(q_4)*(0.099708979*sin(q_4)*(1.0*q_2*sin(q_2) + 1.0*q_1*cos(q_2)*sin(q_2)) - 0.00052231*sin(q_3)*(1.0*q_1*sin(q_2)^2 - 1.0*q_2*cos(q_2)) + 2.61155*sin(q_3)*sin(q_4)*(0.4*q_1*sin(q_2)^2 - 0.4*q_2*cos(q_2)) - 0.099708979*cos(q_3)*cos(q_4)*(1.0*q_1*sin(q_2)^2 - 1.0*q_2*cos(q_2))) - 0.085735584*q_1*cos(q_2)*sin(q_2)) - 1.0*cos(q_3)*(0.00636266901372*cos(q_4)*(1.0*q_2*sin(q_2) + 1.0*q_1*cos(q_2)*sin(q_2)) - 0.065111904*sin(q_3)*(0.4*q_1*sin(q_2)^2 - 0.4*q_2*cos(q_2)) + 0.0011000582042*sin(q_4)*(1.0*q_2*sin(q_2) + 1.0*q_1*cos(q_2)*sin(q_2)) + 0.00220370768768*q_2*sin(q_2) + 0.000142905064*cos(q_3)*(1.0*q_1*sin(q_2)^2 - 1.0*q_2*cos(q_2)) + 0.0610568292028*sin(q_3)*(1.0*q_1*sin(q_2)^2 - 1.0*q_2*cos(q_2)) - 0.00052231*sin(q_3)*sin(q_4)*(0.4*q_1*sin(q_2)^2 - 0.4*q_2*cos(q_2)) + 0.00220370768768*q_1*cos(q_2)*sin(q_2) - 0.0011000582042*cos(q_3)*cos(q_4)*(1.0*q_1*sin(q_2)^2 - 1.0*q_2*cos(q_2)) + 0.00636266901372*cos(q_3)*sin(q_4)*(1.0*q_1*sin(q_2)^2 - 1.0*q_2*cos(q_2)) + 0.137576454*cos(q_4)*sin(q_3)*(0.4*q_1*sin(q_2)^2 - 0.4*q_2*cos(q_2))) - 0.000122603128375*q_2*cos(q_2) - 0.002664500061125*q_2*sin(q_2) - sin(q_3)*(0.065111904*cos(q_3)*(0.4*q_1*sin(q_2)^2 - 0.4*q_2*cos(q_2)) + 1.0*cos(q_4)*(0.0009075152908*cos(q_4)*(1.0*q_2*sin(q_2) + 1.0*q_1*cos(q_2)*sin(q_2)) - 0.137576454*cos(q_3)*(0.4*q_1*sin(q_2)^2 - 0.4*q_2*cos(q_2)) + 0.04949441641494*sin(q_4)*(1.0*q_2*sin(q_2) + 1.0*q_1*cos(q_2)*sin(q_2)) - 0.0011399417958*sin(q_3)*(1.0*q_1*sin(q_2)^2 - 1.0*q_2*cos(q_2)) + 0.099708979*sin(q_3)*sin(q_4)*(0.4*q_1*sin(q_2)^2 - 0.4*q_2*cos(q_2)) - 0.04949441641494*cos(q_3)*cos(q_4)*(1.0*q_1*sin(q_2)^2 - 1.0*q_2*cos(q_2)) + 0.0009075152908*cos(q_3)*sin(q_4)*(1.0*q_1*sin(q_2)^2 - 1.0*q_2*cos(q_2))) - 1.0*sin(q_4)*(0.01524699328022*cos(q_4)*(1.0*q_2*sin(q_2) + 1.0*q_1*cos(q_2)*sin(q_2)) - 0.00052231*cos(q_3)*(0.4*q_1*sin(q_2)^2 - 0.4*q_2*cos(q_2)) - 0.0008524847092*sin(q_4)*(1.0*q_2*sin(q_2) + 1.0*q_1*cos(q_2)*sin(q_2)) + 0.00414266901372*sin(q_3)*(1.0*q_1*sin(q_2)^2 - 1.0*q_2*cos(q_2)) + 0.0008524847092*cos(q_3)*cos(q_4)*(1.0*q_1*sin(q_2)^2 - 1.0*q_2*cos(q_2)) + 0.01524699328022*cos(q_3)*sin(q_4)*(1.0*q_1*sin(q_2)^2 - 1.0*q_2*cos(q_2)) + 0.099708979*cos(q_4)*sin(q_3)*(0.4*q_1*sin(q_2)^2 - 0.4*q_2*cos(q_2))) + 0.000076501784*q_2*sin(q_2) - 0.00695065428736*cos(q_3)*(1.0*q_1*sin(q_2)^2 - 1.0*q_2*cos(q_2)) - 0.000242905064*sin(q_3)*(1.0*q_1*sin(q_2)^2 - 1.0*q_2*cos(q_2)) + 0.000076501784*q_1*cos(q_2)*sin(q_2)) - 0.002664500061125*q_1*cos(q_2)*sin(q_2);
c23=sin(q_3)*(0.000242905064*cos(q_3)*(q_2*sin(q_3) - 1.0*q_1*cos(q_3)*sin(q_2)) - 0.00695065428736*sin(q_3)*(q_2*sin(q_3) - 1.0*q_1*cos(q_3)*sin(q_2)) + 1.0*cos(q_4)*(0.0011399417958*cos(q_3)*(q_2*sin(q_3) - 1.0*q_1*cos(q_3)*sin(q_2)) + 0.0011399417958*sin(q_3)*(q_3 + q_1*cos(q_2)) - 0.04949441641494*cos(q_4)*(1.0*sin(q_3)*(q_2*sin(q_3) - 1.0*q_1*cos(q_3)*sin(q_2)) - 1.0*cos(q_3)*(q_3 + q_1*cos(q_2))) + 0.0009075152908*sin(q_4)*(1.0*sin(q_3)*(q_2*sin(q_3) - 1.0*q_1*cos(q_3)*sin(q_2)) - 1.0*cos(q_3)*(q_3 + q_1*cos(q_2)))) + 0.00695065428736*cos(q_3)*(q_3 + q_1*cos(q_2)) + 1.0*sin(q_4)*(0.00414266901372*cos(q_3)*(q_2*sin(q_3) - 1.0*q_1*cos(q_3)*sin(q_2)) + 0.00414266901372*sin(q_3)*(q_3 + q_1*cos(q_2)) - 0.0008524847092*cos(q_4)*(1.0*sin(q_3)*(q_2*sin(q_3) - 1.0*q_1*cos(q_3)*sin(q_2)) - 1.0*cos(q_3)*(q_3 + q_1*cos(q_2))) - 0.01524699328022*sin(q_4)*(1.0*sin(q_3)*(q_2*sin(q_3) - 1.0*q_1*cos(q_3)*sin(q_2)) - 1.0*cos(q_3)*(q_3 + q_1*cos(q_2)))) + 0.000242905064*sin(q_3)*(q_3 + q_1*cos(q_2))) - 1.0*cos(q_3)*(0.0610568292028*cos(q_3)*(q_2*sin(q_3) - 1.0*q_1*cos(q_3)*sin(q_2)) - 0.000142905064*sin(q_3)*(q_2*sin(q_3) - 1.0*q_1*cos(q_3)*sin(q_2)) + 0.000142905064*cos(q_3)*(q_3 + q_1*cos(q_2)) + 0.0610568292028*sin(q_3)*(q_3 + q_1*cos(q_2)) + 0.0011000582042*cos(q_4)*(1.0*sin(q_3)*(q_2*sin(q_3) - 1.0*q_1*cos(q_3)*sin(q_2)) - 1.0*cos(q_3)*(q_3 + q_1*cos(q_2))) - 0.00636266901372*sin(q_4)*(1.0*sin(q_3)*(q_2*sin(q_3) - 1.0*q_1*cos(q_3)*sin(q_2)) - 1.0*cos(q_3)*(q_3 + q_1*cos(q_2)))) + 0.4*sin(q_3)*(0.065111904*sin(q_3)*(q_2*sin(q_3) - 1.0*q_1*cos(q_3)*sin(q_2)) - 0.065111904*cos(q_3)*(q_3 + q_1*cos(q_2)) - 0.137576454*cos(q_4)*(1.0*sin(q_3)*(q_2*sin(q_3) - 1.0*q_1*cos(q_3)*sin(q_2)) - 1.0*cos(q_3)*(q_3 + q_1*cos(q_2))) + 0.00052231*sin(q_4)*(1.0*sin(q_3)*(q_2*sin(q_3) - 1.0*q_1*cos(q_3)*sin(q_2)) - 1.0*cos(q_3)*(q_3 + q_1*cos(q_2)))) + 0.4*cos(q_3)*(0.065111904*cos(q_3)*(q_2*sin(q_3) - 1.0*q_1*cos(q_3)*sin(q_2)) + 1.0*sin(q_4)*(0.00052231*cos(q_3)*(q_2*sin(q_3) - 1.0*q_1*cos(q_3)*sin(q_2)) + 0.00052231*sin(q_3)*(q_3 + q_1*cos(q_2)) - 0.099708979*cos(q_4)*(1.0*sin(q_3)*(q_2*sin(q_3) - 1.0*q_1*cos(q_3)*sin(q_2)) - 1.0*cos(q_3)*(q_3 + q_1*cos(q_2)))) - cos(q_4)*(0.137576454*cos(q_3)*(q_2*sin(q_3) - 1.0*q_1*cos(q_3)*sin(q_2)) + 0.137576454*sin(q_3)*(q_3 + q_1*cos(q_2)) - 0.099708979*sin(q_4)*(1.0*sin(q_3)*(q_2*sin(q_3) - 1.0*q_1*cos(q_3)*sin(q_2)) - 1.0*cos(q_3)*(q_3 + q_1*cos(q_2)))) + 0.065111904*sin(q_3)*(q_3 + q_1*cos(q_2)));
c24=- sin(q_3)*(1.0*sin(q_4)*(0.0008524847092*sin(q_4)*(cos(q_4)*(q_2*sin(q_3) - 1.0*q_1*cos(q_3)*sin(q_2)) + sin(q_4)*(q_3 + q_1*cos(q_2))) - 0.01524699328022*cos(q_4)*(cos(q_4)*(q_2*sin(q_3) - 1.0*q_1*cos(q_3)*sin(q_2)) + sin(q_4)*(q_3 + q_1*cos(q_2))) + 0.0008524847092*cos(q_4)*(q_2*cos(q_3) - 1.0*q_4 + q_1*sin(q_2)*sin(q_3)) + 0.01524699328022*sin(q_4)*(q_2*cos(q_3) - 1.0*q_4 + q_1*sin(q_2)*sin(q_3))) + 1.0*cos(q_4)*(0.0009075152908*cos(q_4)*(cos(q_4)*(q_2*sin(q_3) - 1.0*q_1*cos(q_3)*sin(q_2)) + sin(q_4)*(q_3 + q_1*cos(q_2))) + 0.04949441641494*sin(q_4)*(cos(q_4)*(q_2*sin(q_3) - 1.0*q_1*cos(q_3)*sin(q_2)) + sin(q_4)*(q_3 + q_1*cos(q_2))) + 0.04949441641494*cos(q_4)*(q_2*cos(q_3) - 1.0*q_4 + q_1*sin(q_2)*sin(q_3)) - 0.0009075152908*sin(q_4)*(q_2*cos(q_3) - 1.0*q_4 + q_1*sin(q_2)*sin(q_3)))) - 0.4*cos(q_3)*(cos(q_4)*(0.099708979*cos(q_4)*(cos(q_4)*(q_2*sin(q_3) - 1.0*q_1*cos(q_3)*sin(q_2)) + sin(q_4)*(q_3 + q_1*cos(q_2))) - 0.099708979*sin(q_4)*(q_2*cos(q_3) - 1.0*q_4 + q_1*sin(q_2)*sin(q_3))) + 1.0*sin(q_4)*(0.099708979*sin(q_4)*(cos(q_4)*(q_2*sin(q_3) - 1.0*q_1*cos(q_3)*sin(q_2)) + sin(q_4)*(q_3 + q_1*cos(q_2))) + 0.099708979*cos(q_4)*(q_2*cos(q_3) - 1.0*q_4 + q_1*sin(q_2)*sin(q_3)))) - 0.4*sin(q_3)*(0.00052231*cos(q_4)*(cos(q_4)*(q_2*sin(q_3) - 1.0*q_1*cos(q_3)*sin(q_2)) + sin(q_4)*(q_3 + q_1*cos(q_2))) + 0.137576454*sin(q_4)*(cos(q_4)*(q_2*sin(q_3) - 1.0*q_1*cos(q_3)*sin(q_2)) + sin(q_4)*(q_3 + q_1*cos(q_2))) + 0.137576454*cos(q_4)*(q_2*cos(q_3) - 1.0*q_4 + q_1*sin(q_2)*sin(q_3)) - 0.00052231*sin(q_4)*(q_2*cos(q_3) - 1.0*q_4 + q_1*sin(q_2)*sin(q_3))) - 1.0*cos(q_3)*(0.00636266901372*cos(q_4)*(cos(q_4)*(q_2*sin(q_3) - 1.0*q_1*cos(q_3)*sin(q_2)) + sin(q_4)*(q_3 + q_1*cos(q_2))) + 0.0011000582042*sin(q_4)*(cos(q_4)*(q_2*sin(q_3) - 1.0*q_1*cos(q_3)*sin(q_2)) + sin(q_4)*(q_3 + q_1*cos(q_2))) + 0.0011000582042*cos(q_4)*(q_2*cos(q_3) - 1.0*q_4 + q_1*sin(q_2)*sin(q_3)) - 0.00636266901372*sin(q_4)*(q_2*cos(q_3) - 1.0*q_4 + q_1*sin(q_2)*sin(q_3)));
c31=0;
c32=0.085735584*sin(q_3)*(0.4*q_1*sin(q_2)^2 - 0.4*q_2*cos(q_2)) - 0.0055242*cos(q_3)*(0.4*q_1*sin(q_2)^2 - 0.4*q_2*cos(q_2)) - 1.0*cos(q_4)*(0.01524699328022*cos(q_4)*(1.0*q_2*sin(q_2) + 1.0*q_1*cos(q_2)*sin(q_2)) - 0.00052231*cos(q_3)*(0.4*q_1*sin(q_2)^2 - 0.4*q_2*cos(q_2)) - 0.0008524847092*sin(q_4)*(1.0*q_2*sin(q_2) + 1.0*q_1*cos(q_2)*sin(q_2)) + 0.00414266901372*sin(q_3)*(1.0*q_1*sin(q_2)^2 - 1.0*q_2*cos(q_2)) + 0.0008524847092*cos(q_3)*cos(q_4)*(1.0*q_1*sin(q_2)^2 - 1.0*q_2*cos(q_2)) + 0.01524699328022*cos(q_3)*sin(q_4)*(1.0*q_1*sin(q_2)^2 - 1.0*q_2*cos(q_2)) + 0.099708979*cos(q_4)*sin(q_3)*(0.4*q_1*sin(q_2)^2 - 0.4*q_2*cos(q_2))) - sin(q_4)*(0.0009075152908*cos(q_4)*(1.0*q_2*sin(q_2) + 1.0*q_1*cos(q_2)*sin(q_2)) - 0.137576454*cos(q_3)*(0.4*q_1*sin(q_2)^2 - 0.4*q_2*cos(q_2)) + 0.04949441641494*sin(q_4)*(1.0*q_2*sin(q_2) + 1.0*q_1*cos(q_2)*sin(q_2)) - 0.0011399417958*sin(q_3)*(1.0*q_1*sin(q_2)^2 - 1.0*q_2*cos(q_2)) + 0.099708979*sin(q_3)*sin(q_4)*(0.4*q_1*sin(q_2)^2 - 0.4*q_2*cos(q_2)) - 0.04949441641494*cos(q_3)*cos(q_4)*(1.0*q_1*sin(q_2)^2 - 1.0*q_2*cos(q_2)) + 0.0009075152908*cos(q_3)*sin(q_4)*(1.0*q_1*sin(q_2)^2 - 1.0*q_2*cos(q_2))) - 0.00373631604328*q_2*sin(q_2) + 0.000216501784*cos(q_3)*(1.0*q_1*sin(q_2)^2 - 1.0*q_2*cos(q_2)) - 0.00234370768768*sin(q_3)*(1.0*q_1*sin(q_2)^2 - 1.0*q_2*cos(q_2)) - 0.00373631604328*q_1*cos(q_2)*sin(q_2);
c33=0.000216501784*cos(q_3)*(q_3 + q_1*cos(q_2)) - 0.000216501784*sin(q_3)*(q_2*sin(q_3) - 1.0*q_1*cos(q_3)*sin(q_2)) - 1.0*cos(q_4)*(0.00414266901372*cos(q_3)*(q_2*sin(q_3) - 1.0*q_1*cos(q_3)*sin(q_2)) + 0.00414266901372*sin(q_3)*(q_3 + q_1*cos(q_2)) - 0.0008524847092*cos(q_4)*(1.0*sin(q_3)*(q_2*sin(q_3) - 1.0*q_1*cos(q_3)*sin(q_2)) - 1.0*cos(q_3)*(q_3 + q_1*cos(q_2))) - 0.01524699328022*sin(q_4)*(1.0*sin(q_3)*(q_2*sin(q_3) - 1.0*q_1*cos(q_3)*sin(q_2)) - 1.0*cos(q_3)*(q_3 + q_1*cos(q_2)))) - 0.00234370768768*cos(q_3)*(q_2*sin(q_3) - 1.0*q_1*cos(q_3)*sin(q_2)) + sin(q_4)*(0.0011399417958*cos(q_3)*(q_2*sin(q_3) - 1.0*q_1*cos(q_3)*sin(q_2)) + 0.0011399417958*sin(q_3)*(q_3 + q_1*cos(q_2)) - 0.04949441641494*cos(q_4)*(1.0*sin(q_3)*(q_2*sin(q_3) - 1.0*q_1*cos(q_3)*sin(q_2)) - 1.0*cos(q_3)*(q_3 + q_1*cos(q_2))) + 0.0009075152908*sin(q_4)*(1.0*sin(q_3)*(q_2*sin(q_3) - 1.0*q_1*cos(q_3)*sin(q_2)) - 1.0*cos(q_3)*(q_3 + q_1*cos(q_2)))) - 0.00234370768768*sin(q_3)*(q_3 + q_1*cos(q_2));
c34=1.0*cos(q_4)*(0.0008524847092*sin(q_4)*(cos(q_4)*(q_2*sin(q_3) - 1.0*q_1*cos(q_3)*sin(q_2)) + sin(q_4)*(q_3 + q_1*cos(q_2))) - 0.01524699328022*cos(q_4)*(cos(q_4)*(q_2*sin(q_3) - 1.0*q_1*cos(q_3)*sin(q_2)) + sin(q_4)*(q_3 + q_1*cos(q_2))) + 0.0008524847092*cos(q_4)*(q_2*cos(q_3) - 1.0*q_4 + q_1*sin(q_2)*sin(q_3)) + 0.01524699328022*sin(q_4)*(q_2*cos(q_3) - 1.0*q_4 + q_1*sin(q_2)*sin(q_3))) - sin(q_4)*(0.0009075152908*cos(q_4)*(cos(q_4)*(q_2*sin(q_3) - 1.0*q_1*cos(q_3)*sin(q_2)) + sin(q_4)*(q_3 + q_1*cos(q_2))) + 0.04949441641494*sin(q_4)*(cos(q_4)*(q_2*sin(q_3) - 1.0*q_1*cos(q_3)*sin(q_2)) + sin(q_4)*(q_3 + q_1*cos(q_2))) + 0.04949441641494*cos(q_4)*(q_2*cos(q_3) - 1.0*q_4 + q_1*sin(q_2)*sin(q_3)) - 0.0009075152908*sin(q_4)*(q_2*cos(q_3) - 1.0*q_4 + q_1*sin(q_2)*sin(q_3)));
c41=0;
c42=0.00636266901372*cos(q_4)*(1.0*q_2*sin(q_2) + 1.0*q_1*cos(q_2)*sin(q_2)) + 0.0011000582042*sin(q_4)*(1.0*q_2*sin(q_2) + 1.0*q_1*cos(q_2)*sin(q_2)) + 0.05712763205872*sin(q_3)*(1.0*q_1*sin(q_2)^2 - 1.0*q_2*cos(q_2)) - 0.00052231*sin(q_3)*sin(q_4)*(0.4*q_1*sin(q_2)^2 - 0.4*q_2*cos(q_2)) - 0.0011000582042*cos(q_3)*cos(q_4)*(1.0*q_1*sin(q_2)^2 - 1.0*q_2*cos(q_2)) + 0.00636266901372*cos(q_3)*sin(q_4)*(1.0*q_1*sin(q_2)^2 - 1.0*q_2*cos(q_2)) + 0.137576454*cos(q_4)*sin(q_3)*(0.4*q_1*sin(q_2)^2 - 0.4*q_2*cos(q_2));
c43=0.05712763205872*cos(q_3)*(q_2*sin(q_3) - 1.0*q_1*cos(q_3)*sin(q_2)) + 0.05712763205872*sin(q_3)*(q_3 + q_1*cos(q_2)) + 0.0011000582042*cos(q_4)*(1.0*sin(q_3)*(q_2*sin(q_3) - 1.0*q_1*cos(q_3)*sin(q_2)) - 1.0*cos(q_3)*(q_3 + q_1*cos(q_2))) - 0.00636266901372*sin(q_4)*(1.0*sin(q_3)*(q_2*sin(q_3) - 1.0*q_1*cos(q_3)*sin(q_2)) - 1.0*cos(q_3)*(q_3 + q_1*cos(q_2)));
c44=0.00636266901372*cos(q_4)*(cos(q_4)*(q_2*sin(q_3) - 1.0*q_1*cos(q_3)*sin(q_2)) + sin(q_4)*(q_3 + q_1*cos(q_2))) + 0.0011000582042*sin(q_4)*(cos(q_4)*(q_2*sin(q_3) - 1.0*q_1*cos(q_3)*sin(q_2)) + sin(q_4)*(q_3 + q_1*cos(q_2))) + 0.0011000582042*cos(q_4)*(q_2*cos(q_3) - 1.0*q_4 + q_1*sin(q_2)*sin(q_3)) - 0.00636266901372*sin(q_4)*(q_2*cos(q_3) - 1.0*q_4 + q_1*sin(q_2)*sin(q_3));

C=[c11 c12 c13 c14;c21 c22 c23 c24;c31 c32 c33 c34;c41 c42 c43 c44];
 

M_11=m22*m33*m44 + m23*m34*m42 + m24*m32*m43 - m24*m33*m42 - m23*m32*m44 -m22*m34*m43;
M_12=-m12*m33*m44 - m13*m34*m42 - m14*m32*m43 + m14*m33*m42 + m13*m32*m44 + m12*m34*m43;
M_13=m12*m23*m44 + m13*m24*m42 + m14*m22*m43 - m14*m23*m42 - m13*m22*m44 - m12*m24*m43;
M_14=-m12*m23*m34 - m13*m24*m32 - m14*m22*m33 + m14*m23*m32 + m13*m22*m34 + m12*m24*m33;
M_21=-m21*m33*m44 - m23*m34*m41 - m24*m31*m43 + m24*m33*m41 + m23*m31*m44 + m21*m34*m43;
M_22=m11*m33*m44 + m13*m34*m41 + m14*m31*m43 - m14*m33*m41 - m13*m31*m44 - m11*m34*m43;
M_23=-m11*m23*m44 - m13*m24*m41 - m14*m21*m43 + m14*m23*m41 + m13*m21*m44 + m11*m24*m43;
M_24=m11*m23*m34 + m13*m24*m31 + m14*m21*m33 - m14*m23*m31 - m13*m21*m34 - m11*m24*m33;
M_31=m21*m32*m44+m22*m34*m41+m24*m31*m42-m24*m32*m41-m22*m31*m44-m21*m34*m42;
M_32=-m11*m32*m44-m12*m34*m41-m14*m31*m42+m14*m32*m41+m12*m31*m44+m11*m34*m42;
M_33=m11*m22*m44+m12*m24*m41+m14*m21*m42-m14*m22*m41-m12*m21*m44-m11*m24*m42;
M_34=-m11*m22*m34-m12*m24*m31-m14*m21*m32+m14*m22*m31+m12*m21*m34+m11*m24*m32;
M_41=-m21*m32*m43-m22*m33*m41-m23*m31*m42+m23*m32*m41+m22*m31*m43+m21*m33*m42;
M_42=m11*m32*m43+m12*m33*m41+m13*m31*m42-m13*m32*m41-m12*m31*m43-m11*m33*m42;
M_43=-m11*m22*m43-m12*m23*m41-m13*m21*m42+m13*m22*m41+m12*m21*m43+m11*m23*m42;
M_44=m11*m22*m33+m12*m23*m31+m13*m21*m32-m13*m22*m31-m12*m21*m33-m11*m23*m32;


det_M = m11*m22*m33*m44 + m11*m23*m34*m42 + m11*m24*m32*m43 - m11*m24*m33*m42 - m11*m23*m32*m44 - m11*m22*m34*m43 - m12*m21*m33*m44 - m13*m21*m34*m42 - m14*m21*m32*m43 + m14*m21*m33*m42 + m13*m21*m32*m44 + m12*m21*m34*m43 + m12*m23*m31*m44 + m13*m24*m31*m42 + m14*m22*m31*m43 - m14*m23*m31*m42 - m13*m22*m31*m44 - m12*m24*m31*m43 - m12*m23*m34*m41 - m13*m24*m32*m41 - m14*m22*m33*m41 + m14*m23*m32*m41 + m13*m22*m34*m41 + m12*m24*m33*m41;

inv_M=[M_11 M_12 M_13 M_14;M_21 M_22 M_23 M_24;M_31 M_32 M_33 M_34;M_41 M_42 M_43 M_44]/det_M;

q_ddot = inv_M*(torque - C*q_dot);

== matlab function kuka_sim/MATLAB Function ==
  data: q input; q_1 output; q_dot input; q_ddot input; q_1_dot output; q_2 output; q_2_dot output; q_3 output; q_3_dot output; q_4 output; q_4_dot output; q_1_ddot output; q_2_ddot output; q_3_ddot output; q_4_ddot output
function [q_1,q_1_dot,q_2,q_2_dot,q_3,q_3_dot,q_4,q_4_dot,q_1_ddot,q_2_ddot,q_3_ddot,q_4_ddot] = fcn(q,q_dot,q_ddot)
%#codegen

q_1 = q(1);
q_2 = q(2);
q_3 = q(3);
q_4 = q(4);

q_1_dot = q_dot(1);
q_2_dot = q_dot(2);
q_3_dot = q_dot(3);
q_4_dot = q_dot(4);

q_1_ddot = q_ddot(1);
q_2_ddot = q_ddot(2);
q_3_ddot = q_ddot(3);
q_4_ddot = q_ddot(4);

== matlab function kuka_sim/MATLAB Function1 ==
  data: q_1 input; J output; q_1_dot input; q_2 input; q_2_dot input; q_3 input; q_3_dot input; q_4 input; q_4_dot input; q_1_ddot input; q_2_ddot input; q_3_ddot input; q_4_ddot input; J_dot output; X_dot output; X_ddot output
function [J,J_dot,X_dot,X_ddot] = fcn(q_1,q_1_dot,q_2,q_2_dot,q_3,q_3_dot,q_4,q_4_dot,q_1_ddot,q_2_ddot,q_3_ddot,q_4_ddot)

j1=[ 0.4*sin(q_1)*sin(q_2), -0.4*cos(q_1)*cos(q_2), 0, 0];
j2=[ -0.4*cos(q_1)*sin(q_2), -0.4*cos(q_2)*sin(q_1), 0, 0];
j3=[ 0, - 0.4*cos(q_1)^2*sin(q_2) - 0.4*sin(q_1)^2*sin(q_2), 0, 0];
j4=[ 0, 1.0*sin(q_1), -1.0*cos(q_1)*sin(q_2), - 1.0*cos(q_3)*sin(q_1) - 1.0*cos(q_1)*cos(q_2)*sin(q_3)];
j5=[ 0, -1.0*cos(q_1), -1.0*sin(q_1)*sin(q_2), 1.0*cos(q_1)*cos(q_3) - 1.0*cos(q_2)*sin(q_1)*sin(q_3)];
j6=[ 1.0, 0, 1.0*cos(q_2), -1.0*sin(q_2)*sin(q_3)];

J=[j1;j2;j3;j4;j5;j6];
% J=[j1;j2;j3];

j1_dot=[ 0.4*q_1_dot*cos(q_1)*sin(q_2) + 0.4*q_2_dot*cos(q_2)*sin(q_1), 0.4*q_1_dot*cos(q_2)*sin(q_1) + 0.4*q_2_dot*cos(q_1)*sin(q_2), 0, 0];
j2_dot=[ 0.4*q_1_dot*sin(q_1)*sin(q_2) - 0.4*q_2_dot*cos(q_1)*cos(q_2), 0.4*q_2_dot*sin(q_1)*sin(q_2) - 0.4*q_1_dot*cos(q_1)*cos(q_2), 0, 0];
j3_dot=[ 0, -q_2_dot*(0.4*cos(q_1)^2*cos(q_2) + 0.4*cos(q_2)*sin(q_1)^2), 0, 0];
j4_dot=[ 0, 1.0*q_1_dot*cos(q_1), 1.0*q_1_dot*sin(q_1)*sin(q_2) - 1.0*q_2_dot*cos(q_1)*cos(q_2), q_3_dot*(1.0*sin(q_1)*sin(q_3) - 1.0*cos(q_1)*cos(q_2)*cos(q_3)) - q_1_dot*(1.0*cos(q_1)*cos(q_3) - 1.0*cos(q_2)*sin(q_1)*sin(q_3)) + 1.0*q_2_dot*cos(q_1)*sin(q_2)*sin(q_3)];
j5_dot=[ 0, 1.0*q_1_dot*sin(q_1), - 1.0*q_1_dot*cos(q_1)*sin(q_2) - 1.0*q_2_dot*cos(q_2)*sin(q_1), 1.0*q_2_dot*sin(q_1)*sin(q_2)*sin(q_3) - q_3_dot*(1.0*cos(q_1)*sin(q_3) + 1.0*cos(q_2)*cos(q_3)*sin(q_1)) - q_1_dot*(1.0*cos(q_3)*sin(q_1) + 1.0*cos(q_1)*cos(q_2)*sin(q_3))];
j6_dot=[ 0, 0, -1.0*q_2_dot*sin(q_2), - 1.0*q_2_dot*cos(q_2)*sin(q_3) - 1.0*q_3_dot*cos(q_3)*sin(q_2)];

J_dot=[j1_dot;j2_dot;j3_dot;j4_dot;j5_dot;j6_dot];
% J_dot=[j1_dot;j2_dot;j3_dot];

X_dot = J*[q_1_dot ; q_2_dot ; q_3_dot ; q_4_dot];
X_ddot = J_dot*[q_1_dot ; q_2_dot ; q_3_dot;q_4_dot] + J*[q_1_ddot ; q_2_ddot ; q_3_ddot; q_4_ddot];
